simulink model "c00006M_harness"  (R2018a)
settings: Solver=ode3  StartTime=0.0  StopTime=10.0  RelTol=1e-3  EnableMultiTasking=on
undefined symbols (not defined in the file): b, DiscIntNeverNeededParam, J, K, L, PosMinimaW3, R, sigbuilder_block
(part 1 of 42)
settings Model: Creator=aarrieta  LastModifiedBy=umarkiegi
settings DataIOCC: LimitDataPoints=on  SaveFormat=Array
settings OptimizationCC: LifeSpan=inf
settings DebuggingCC: UnderspecifiedInitializationDetection=Classic  MergeDetectMultiDrivingBlocksExec=none  SolverPrmCheckMsg=warning  StateNameClashWarn=warning  SFUnexpectedBacktrackingDiag=warning  SFNoUnconditionalDefaultTransitionDiag=warning  SFExecutionAtInitializationDiag=none
settings HardwareCC: ProdBitPerPointer=32  ProdBitPerSizeT=32  ProdBitPerPtrDiffT=32  ProdLargestAtomicFloat=None  ProdIntDivRoundTo=Undefined  ProdEndianess=Unspecified  ProdWordSize=32  ProdHWDeviceType=32-bit Generic
settings ModelReferenceCC: PropagateSignalLabelsOutOfModel=off
settings CodeAppCC: StateflowObjectComments=on
settings GRTTargetCC: TargetLangStandard=C89/C90 (ANSI)  GeneratePreprocessorConditionals=Disable all
settings ConfigComp: CovMetricSettings=dw  CovHtmlReporting=on  CovSaveCumulativeToWorkspaceVar=on  CovSaveSingleToWorkspaceVar=on  CovExternalEMLEnable=off  DVMaxTestCaseSteps=20  DVTestSuiteOptimization=CombinedObjectives (Nonlinear Extended)  DVDetectFloatOverflow=off

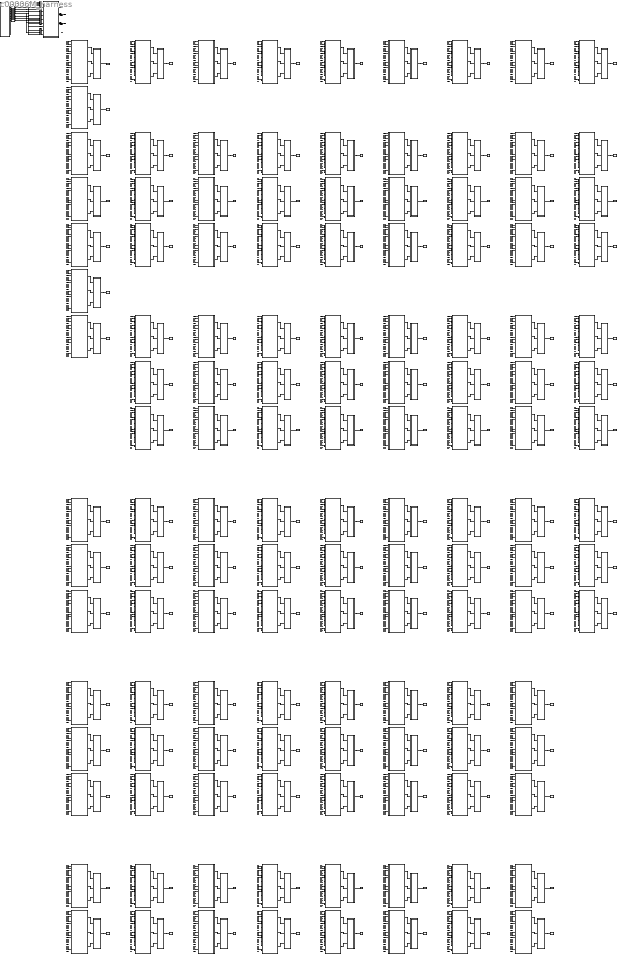
== system c00006M_harness ==
  CPSUT : Subsystem
  Eval : Subsystem
  Eval1 : Subsystem
  Eval10 : Subsystem
  Eval100 : Subsystem
  Eval102 : Subsystem
  Eval103 : Subsystem
  Eval104 : Subsystem
  Eval106 : Subsystem
  Eval107 : Subsystem
  Eval108 : Subsystem
  Eval11 : Subsystem
  Eval110 : Subsystem
  Eval111 : Subsystem
  Eval112 : Subsystem
  Eval114 : Subsystem
  Eval115 : Subsystem
  Eval116 : Subsystem
  Eval118 : Subsystem
  Eval119 : Subsystem
  Eval12 : Subsystem
  Eval120 : Subsystem
  Eval122 : Subsystem
  Eval123 : Subsystem
  Eval124 : Subsystem
  Eval126 : Subsystem
  Eval127 : Subsystem
  Eval128 : Subsystem
  Eval130 : Subsystem
  Eval131 : Subsystem
  Eval132 : Subsystem
  Eval134 : Subsystem
  Eval135 : Subsystem
  Eval136 : Subsystem
  Eval138 : Subsystem
  Eval139 : Subsystem
  Eval14 : Subsystem
  Eval140 : Subsystem
  Eval142 : Subsystem
  Eval143 : Subsystem
  Eval144 : Subsystem
  Eval146 : Subsystem
  Eval147 : Subsystem
  Eval148 : Subsystem
  Eval15 : Subsystem
  Eval150 : Subsystem
  Eval151 : Subsystem
  Eval152 : Subsystem
  Eval154 : Subsystem
  Eval155 : Subsystem
  Eval156 : Subsystem
  Eval158 : Subsystem
  Eval159 : Subsystem
  Eval16 : Subsystem
  Eval160 : Subsystem
  Eval162 : Subsystem
  Eval163 : Subsystem
  Eval164 : Subsystem
  Eval166 : Subsystem
  Eval167 : Subsystem
  Eval168 : Subsystem
  Eval170 : Subsystem
  Eval171 : Subsystem
  Eval172 : Subsystem
  Eval18 : Subsystem
  Eval19 : Subsystem
  Eval2 : Subsystem
  Eval20 : Subsystem
  Eval22 : Subsystem
  Eval23 : Subsystem
  Eval24 : Subsystem
  Eval26 : Subsystem
  Eval27 : Subsystem
  Eval28 : Subsystem
  Eval3 : Subsystem
  Eval30 : Subsystem
  Eval31 : Subsystem
  Eval32 : Subsystem
  Eval34 : Subsystem
  Eval35 : Subsystem
  Eval36 : Subsystem
  Eval38 : Subsystem
  Eval39 : Subsystem
  Eval4 : Subsystem
  Eval40 : Subsystem
  Eval42 : Subsystem
  Eval43 : Subsystem
  Eval44 : Subsystem
  Eval46 : Subsystem
  Eval47 : Subsystem
  Eval48 : Subsystem
  Eval5 : Subsystem
  Eval50 : Subsystem
  Eval51 : Subsystem
  Eval52 : Subsystem
  Eval54 : Subsystem
  Eval55 : Subsystem
  Eval56 : Subsystem
  Eval58 : Subsystem
  Eval59 : Subsystem
  Eval6 : Subsystem
  Eval60 : Subsystem
  Eval62 : Subsystem
  Eval63 : Subsystem
  Eval64 : Subsystem
  Eval66 : Subsystem
  Eval67 : Subsystem
  Eval68 : Subsystem
  Eval70 : Subsystem
  Eval71 : Subsystem
  Eval72 : Subsystem
  Eval74 : Subsystem
  Eval75 : Subsystem
  Eval76 : Subsystem
  Eval78 : Subsystem
  Eval79 : Subsystem
  Eval80 : Subsystem
  Eval82 : Subsystem
  Eval83 : Subsystem
  Eval84 : Subsystem
  Eval86 : Subsystem
  Eval87 : Subsystem
  Eval88 : Subsystem
  Eval90 : Subsystem
  Eval91 : Subsystem
  Eval92 : Subsystem
  Eval94 : Subsystem
  Eval95 : Subsystem
  Eval96 : Subsystem
  Eval98 : Subsystem
  Eval99 : Subsystem
  Inputs : Subsystem  Tag=STV Subsys  LoadFcn=sigbuilder_block('load');  StartFcn=sigbuilder_block('start');  StopFcn=sigbuilder_block('stop');  ClipboardFcn=sigbuilder_block('clipboard');  mask(Sigbuilder block){tuvar=[0:10]}
      mask init:
      | if ~strcmp(get_param(bdroot(gcb),'SimulationStatus'),'stopped'),tuvar = sigbuilder_block('maskInit'); end
      settings: CopyFcn=sigbuilder_block('copy');  DeleteFcn=sigbuilder_block('delete');  ModelCloseFcn=sigbuilder_block('modelClose');  PreSaveFcn=sigbuilder_block('preSave');  PauseFcn=sigbuilder_block('pause');  ContinueFcn=sigbuilder_block('continue');  NameChangeFcn=sigbuilder_block('namechange');  OpenFcn=sigbuilder_block('open');  CloseFcn=sigbuilder_block('close');
      mask Display: plot(0, 0, 100, 100,[2, 2, 32, 32, 2], [68, 8, 8, 68, 68],[32, 2], [38, 38], [32, 19, 2],[53, 60, 44], [32, 17, 17, 2],[16, 16, 31, 31]);txt = getActiveGroup(gcbh);text(2, 100, txt,'verticalAlignment', 'top');
  M001 : Subsystem
  M002 : Subsystem
  M003 : Subsystem
  M004 : Subsystem
  M005 : Subsystem
  M006 : Subsystem
  M007 : Subsystem
  M011 : Subsystem
  M012 : Subsystem
  M013 : Subsystem
  M015 : Subsystem
  M016 : Subsystem
  M017 : Subsystem
  M019 : Subsystem
  M020 : Subsystem
  M021 : Subsystem
  M023 : Subsystem
  M024 : Subsystem
  M025 : Subsystem
  M027 : Subsystem
  M028 : Subsystem
  M029 : Subsystem
  M031 : Subsystem
  M032 : Subsystem
  M033 : Subsystem
  M035 : Subsystem
  M036 : Subsystem
  M037 : Subsystem
  M039 : Subsystem
  M040 : Subsystem
  M041 : Subsystem
  M043 : Subsystem
  M044 : Subsystem
  M045 : Subsystem
  M047 : Subsystem
  M048 : Subsystem
  M049 : Subsystem
  M051 : Subsystem
  M052 : Subsystem
  M053 : Subsystem
  M055 : Subsystem
  M056 : Subsystem
  M057 : Subsystem
  M059 : Subsystem
  M060 : Subsystem
  M061 : Subsystem
  M063 : Subsystem
  M064 : Subsystem
  M065 : Subsystem
  M067 : Subsystem
  M068 : Subsystem
  M069 : Subsystem
  M071 : Subsystem
  M072 : Subsystem
  M073 : Subsystem
  M075 : Subsystem
  M076 : Subsystem
  M077 : Subsystem
  M079 : Subsystem
  M080 : Subsystem
  M081 : Subsystem
  M083 : Subsystem
  M084 : Subsystem
  M085 : Subsystem
  M087 : Subsystem
  M088 : Subsystem
  M089 : Subsystem
  M091 : Subsystem
  M092 : Subsystem
  M093 : Subsystem
  M095 : Subsystem
  M096 : Subsystem
  M097 : Subsystem
  M099 : Subsystem
  M100 : Subsystem
  M101 : Subsystem
  M103 : Subsystem
  M104 : Subsystem
  M105 : Subsystem
  M107 : Subsystem
  M108 : Subsystem
  M109 : Subsystem
  M111 : Subsystem
  M112 : Subsystem
  M113 : Subsystem
  M115 : Subsystem
  M116 : Subsystem
  M117 : Subsystem
  M119 : Subsystem
  M120 : Subsystem
  M121 : Subsystem
  M123 : Subsystem
  M124 : Subsystem
  M125 : Subsystem
  M127 : Subsystem
  M128 : Subsystem
  M129 : Subsystem
  M131 : Subsystem
  M132 : Subsystem
  M133 : Subsystem
  M135 : Subsystem
  M136 : Subsystem
  M137 : Subsystem
  M139 : Subsystem
  M140 : Subsystem
  M141 : Subsystem
  M143 : Subsystem
  M144 : Subsystem
  M145 : Subsystem
  M147 : Subsystem
  M148 : Subsystem
  M149 : Subsystem
  M151 : Subsystem
  M152 : Subsystem
  M153 : Subsystem
  M155 : Subsystem
  M156 : Subsystem
  M157 : Subsystem
  M159 : Subsystem
  M160 : Subsystem
  M161 : Subsystem
  M163 : Subsystem
  M164 : Subsystem
  M165 : Subsystem
  M167 : Subsystem
  M168 : Subsystem
  M169 : Subsystem
  M171 : Subsystem
  M172 : Subsystem
  M173 : Subsystem
  To Workspace : ToWorkspace  VariableName=mutant001  SampleTime=-1
  To Workspace1 : ToWorkspace  VariableName=mutant002  SampleTime=-1
  To Workspace10 : ToWorkspace  VariableName=mutant011  SampleTime=-1
  To Workspace100 : ToWorkspace  VariableName=mutant101  SampleTime=-1
  To Workspace102 : ToWorkspace  VariableName=mutant103  SampleTime=-1
  To Workspace103 : ToWorkspace  VariableName=mutant104  SampleTime=-1
  To Workspace104 : ToWorkspace  VariableName=mutant105  SampleTime=-1
  To Workspace106 : ToWorkspace  VariableName=mutant107  SampleTime=-1
  To Workspace107 : ToWorkspace  VariableName=mutant108  SampleTime=-1
  To Workspace108 : ToWorkspace  VariableName=mutant109  SampleTime=-1
  To Workspace11 : ToWorkspace  VariableName=mutant012  SampleTime=-1
  To Workspace110 : ToWorkspace  VariableName=mutant111  SampleTime=-1
  To Workspace111 : ToWorkspace  VariableName=mutant112  SampleTime=-1
  To Workspace112 : ToWorkspace  VariableName=mutant113  SampleTime=-1
  To Workspace114 : ToWorkspace  VariableName=mutant115  SampleTime=-1
  To Workspace115 : ToWorkspace  VariableName=mutant116  SampleTime=-1
  To Workspace116 : ToWorkspace  VariableName=mutant117  SampleTime=-1
  To Workspace118 : ToWorkspace  VariableName=mutant119  SampleTime=-1
  To Workspace119 : ToWorkspace  VariableName=mutant120  SampleTime=-1
  To Workspace12 : ToWorkspace  VariableName=mutant013  SampleTime=-1
  To Workspace120 : ToWorkspace  VariableName=mutant121  SampleTime=-1
  To Workspace122 : ToWorkspace  VariableName=mutant123  SampleTime=-1
  To Workspace123 : ToWorkspace  VariableName=mutant124  SampleTime=-1
  To Workspace124 : ToWorkspace  VariableName=mutant125  SampleTime=-1
  To Workspace126 : ToWorkspace  VariableName=mutant127  SampleTime=-1
  To Workspace127 : ToWorkspace  VariableName=mutant128  SampleTime=-1
  To Workspace128 : ToWorkspace  VariableName=mutant129  SampleTime=-1
  To Workspace130 : ToWorkspace  VariableName=mutant131  SampleTime=-1
  To Workspace131 : ToWorkspace  VariableName=mutant132  SampleTime=-1
  To Workspace132 : ToWorkspace  VariableName=mutant133  SampleTime=-1
  To Workspace134 : ToWorkspace  VariableName=mutant135  SampleTime=-1
  To Workspace135 : ToWorkspace  VariableName=mutant136  SampleTime=-1
  To Workspace136 : ToWorkspace  VariableName=mutant137  SampleTime=-1
  To Workspace138 : ToWorkspace  VariableName=mutant139  SampleTime=-1
  To Workspace139 : ToWorkspace  VariableName=mutant140  SampleTime=-1
  To Workspace14 : ToWorkspace  VariableName=mutant015  SampleTime=-1
  To Workspace140 : ToWorkspace  VariableName=mutant141  SampleTime=-1
  To Workspace142 : ToWorkspace  VariableName=mutant143  SampleTime=-1
  To Workspace143 : ToWorkspace  VariableName=mutant144  SampleTime=-1
  To Workspace144 : ToWorkspace  VariableName=mutant145  SampleTime=-1
  To Workspace146 : ToWorkspace  VariableName=mutant147  SampleTime=-1
  To Workspace147 : ToWorkspace  VariableName=mutant148  SampleTime=-1
  To Workspace148 : ToWorkspace  VariableName=mutant149  SampleTime=-1
  To Workspace15 : ToWorkspace  VariableName=mutant016  SampleTime=-1
  To Workspace150 : ToWorkspace  VariableName=mutant151  SampleTime=-1
  To Workspace151 : ToWorkspace  VariableName=mutant152  SampleTime=-1
  To Workspace152 : ToWorkspace  VariableName=mutant153  SampleTime=-1
  To Workspace154 : ToWorkspace  VariableName=mutant155  SampleTime=-1
  To Workspace155 : ToWorkspace  VariableName=mutant156  SampleTime=-1
  To Workspace156 : ToWorkspace  VariableName=mutant157  SampleTime=-1
  To Workspace158 : ToWorkspace  VariableName=mutant159  SampleTime=-1
  To Workspace159 : ToWorkspace  VariableName=mutant160  SampleTime=-1
  To Workspace16 : ToWorkspace  VariableName=mutant017  SampleTime=-1
  To Workspace160 : ToWorkspace  VariableName=mutant161  SampleTime=-1
  To Workspace162 : ToWorkspace  VariableName=mutant163  SampleTime=-1
  To Workspace163 : ToWorkspace  VariableName=mutant164  SampleTime=-1
  To Workspace164 : ToWorkspace  VariableName=mutant165  SampleTime=-1
  To Workspace166 : ToWorkspace  VariableName=mutant167  SampleTime=-1
  To Workspace167 : ToWorkspace  VariableName=mutant168  SampleTime=-1
  To Workspace168 : ToWorkspace  VariableName=mutant169  SampleTime=-1
  To Workspace170 : ToWorkspace  VariableName=mutant171  SampleTime=-1
  To Workspace171 : ToWorkspace  VariableName=mutant172  SampleTime=-1
  To Workspace172 : ToWorkspace  VariableName=mutant173  SampleTime=-1
  To Workspace18 : ToWorkspace  VariableName=mutant019  SampleTime=-1
  To Workspace19 : ToWorkspace  VariableName=mutant020  SampleTime=-1
  To Workspace2 : ToWorkspace  VariableName=mutant003  SampleTime=-1
  To Workspace20 : ToWorkspace  VariableName=mutant021  SampleTime=-1
  To Workspace22 : ToWorkspace  VariableName=mutant023  SampleTime=-1
  To Workspace23 : ToWorkspace  VariableName=mutant024  SampleTime=-1
  To Workspace24 : ToWorkspace  VariableName=mutant025  SampleTime=-1
  To Workspace26 : ToWorkspace  VariableName=mutant027  SampleTime=-1
  To Workspace27 : ToWorkspace  VariableName=mutant028  SampleTime=-1
  To Workspace28 : ToWorkspace  VariableName=mutant029  SampleTime=-1
  To Workspace3 : ToWorkspace  VariableName=mutant004  SampleTime=-1
  To Workspace30 : ToWorkspace  VariableName=mutant031  SampleTime=-1
  To Workspace31 : ToWorkspace  VariableName=mutant032  SampleTime=-1
  To Workspace32 : ToWorkspace  VariableName=mutant033  SampleTime=-1
  To Workspace34 : ToWorkspace  VariableName=mutant035  SampleTime=-1
  To Workspace35 : ToWorkspace  VariableName=mutant036  SampleTime=-1
  To Workspace36 : ToWorkspace  VariableName=mutant037  SampleTime=-1
  To Workspace38 : ToWorkspace  VariableName=mutant039  SampleTime=-1
  To Workspace39 : ToWorkspace  VariableName=mutant040  SampleTime=-1
  To Workspace4 : ToWorkspace  VariableName=mutant005  SampleTime=-1
  To Workspace40 : ToWorkspace  VariableName=mutant041  SampleTime=-1
  To Workspace42 : ToWorkspace  VariableName=mutant043  SampleTime=-1
  To Workspace43 : ToWorkspace  VariableName=mutant044  SampleTime=-1
  To Workspace44 : ToWorkspace  VariableName=mutant045  SampleTime=-1
  To Workspace46 : ToWorkspace  VariableName=mutant047  SampleTime=-1
  To Workspace47 : ToWorkspace  VariableName=mutant048  SampleTime=-1
  To Workspace48 : ToWorkspace  VariableName=mutant049  SampleTime=-1
  To Workspace5 : ToWorkspace  VariableName=mutant006  SampleTime=-1
  To Workspace50 : ToWorkspace  VariableName=mutant051  SampleTime=-1
  To Workspace51 : ToWorkspace  VariableName=mutant052  SampleTime=-1
  To Workspace52 : ToWorkspace  VariableName=mutant053  SampleTime=-1
  To Workspace54 : ToWorkspace  VariableName=mutant055  SampleTime=-1
  To Workspace55 : ToWorkspace  VariableName=mutant056  SampleTime=-1
  To Workspace56 : ToWorkspace  VariableName=mutant057  SampleTime=-1
  To Workspace58 : ToWorkspace  VariableName=mutant059  SampleTime=-1
  To Workspace59 : ToWorkspace  VariableName=mutant060  SampleTime=-1
  To Workspace6 : ToWorkspace  VariableName=mutant007  SampleTime=-1
  To Workspace60 : ToWorkspace  VariableName=mutant061  SampleTime=-1
  To Workspace62 : ToWorkspace  VariableName=mutant063  SampleTime=-1
  To Workspace63 : ToWorkspace  VariableName=mutant064  SampleTime=-1
  To Workspace64 : ToWorkspace  VariableName=mutant065  SampleTime=-1
  To Workspace66 : ToWorkspace  VariableName=mutant067  SampleTime=-1
  To Workspace67 : ToWorkspace  VariableName=mutant068  SampleTime=-1
  To Workspace68 : ToWorkspace  VariableName=mutant069  SampleTime=-1
  To Workspace70 : ToWorkspace  VariableName=mutant071  SampleTime=-1
  To Workspace71 : ToWorkspace  VariableName=mutant072  SampleTime=-1
  To Workspace72 : ToWorkspace  VariableName=mutant073  SampleTime=-1
  To Workspace74 : ToWorkspace  VariableName=mutant075  SampleTime=-1
  To Workspace75 : ToWorkspace  VariableName=mutant076  SampleTime=-1
  To Workspace76 : ToWorkspace  VariableName=mutant077  SampleTime=-1
  To Workspace78 : ToWorkspace  VariableName=mutant079  SampleTime=-1
  To Workspace79 : ToWorkspace  VariableName=mutant080  SampleTime=-1
  To Workspace80 : ToWorkspace  VariableName=mutant081  SampleTime=-1
  To Workspace82 : ToWorkspace  VariableName=mutant083  SampleTime=-1
  To Workspace83 : ToWorkspace  VariableName=mutant084  SampleTime=-1
  To Workspace84 : ToWorkspace  VariableName=mutant085  SampleTime=-1
  To Workspace86 : ToWorkspace  VariableName=mutant087  SampleTime=-1
  To Workspace87 : ToWorkspace  VariableName=mutant088  SampleTime=-1
  To Workspace88 : ToWorkspace  VariableName=mutant089  SampleTime=-1
  To Workspace90 : ToWorkspace  VariableName=mutant091  SampleTime=-1
  To Workspace91 : ToWorkspace  VariableName=mutant092  SampleTime=-1
  To Workspace92 : ToWorkspace  VariableName=mutant093  SampleTime=-1
  To Workspace94 : ToWorkspace  VariableName=mutant095  SampleTime=-1
  To Workspace95 : ToWorkspace  VariableName=mutant096  SampleTime=-1
  To Workspace96 : ToWorkspace  VariableName=mutant097  SampleTime=-1
  To Workspace98 : ToWorkspace  VariableName=mutant099  SampleTime=-1
  To Workspace99 : ToWorkspace  VariableName=mutant100  SampleTime=-1
  dtc_CW3C : DataTypeConversion
  dtc_DW1 : DataTypeConversion
  dtc_DW2 : DataTypeConversion
  dtc_DW3 : DataTypeConversion
  dtc_O1 : DataTypeConversion
  dtc_O2 : DataTypeConversion
  dtc_O3 : DataTypeConversion
  dtc_P1W2 : DataTypeConversion
  dtc_P2W3 : DataTypeConversion
  W1Pos : Outport
  W2Pos : Outport  Port=2
  W3Pos : Outport  Port=3
  tag scope: out1=global, out2=global, out3=global, out4=global
  wires:
  CPSUT/2(W2Pos) -> [out2], W2Pos/1
  CPSUT/3(W3Pos) -> W3Pos/1, [out3]
  [in1] -> M001/1(DW1)
  [in2] -> M001/2(DW2)
  [in3] -> M001/3(DW3)
  [in5] -> M001/4(P1W2)
  [in6] -> M001/5(P2W3)
  [in10] -> M001/6(O1)
  [in11] -> M001/7(O2)
  [in12] -> M001/8(O3)
  [in17] -> M001/9(CW3C)
  CPSUT/1(W1Pos) -> [out1], W1Pos/1
  M001/1(W1Pos) -> Eval/1(In1)
  M001/2(W2Pos) -> Eval/2(In2)
  M001/3(W3Pos) -> Eval/3(In3)
  Eval/1(Out1) -> To Workspace/1
  [in1] -> M002/1(DW1)
  [in2] -> M002/2(DW2)
  [in3] -> M002/3(DW3)
  [in5] -> M002/4(P1W2)
  [in6] -> M002/5(P2W3)
  [in10] -> M002/6(O1)
  [in11] -> M002/7(O2)
  [in12] -> M002/8(O3)
  [in17] -> M002/9(CW3C)
  M002/1(W1Pos) -> Eval1/1(In1)
  M002/2(W2Pos) -> Eval1/2(In2)
  M002/3(W3Pos) -> Eval1/3(In3)
  Eval1/1(Out1) -> To Workspace1/1
  [in1] -> M003/1(DW1)
  [in2] -> M003/2(DW2)
  [in3] -> M003/3(DW3)
  [in5] -> M003/4(P1W2)
  [in6] -> M003/5(P2W3)
  [in10] -> M003/6(O1)
  [in11] -> M003/7(O2)
  [in12] -> M003/8(O3)
  [in17] -> M003/9(CW3C)
  M003/1(W1Pos) -> Eval2/1(In1)
  M003/2(W2Pos) -> Eval2/2(In2)
  M003/3(W3Pos) -> Eval2/3(In3)
  Eval2/1(Out1) -> To Workspace2/1
  [in1] -> M004/1(DW1)
  [in2] -> M004/2(DW2)
  [in3] -> M004/3(DW3)
  [in5] -> M004/4(P1W2)
  [in6] -> M004/5(P2W3)
  [in10] -> M004/6(O1)
  [in11] -> M004/7(O2)
  [in12] -> M004/8(O3)
  [in17] -> M004/9(CW3C)
  M004/1(W1Pos) -> Eval3/1(In1)
  M004/2(W2Pos) -> Eval3/2(In2)
  M004/3(W3Pos) -> Eval3/3(In3)
  Eval3/1(Out1) -> To Workspace3/1
  [in1] -> M005/1(DW1)
  [in2] -> M005/2(DW2)
  [in3] -> M005/3(DW3)
  [in5] -> M005/4(P1W2)
  [in6] -> M005/5(P2W3)
  [in10] -> M005/6(O1)
  [in11] -> M005/7(O2)
  [in12] -> M005/8(O3)
  [in17] -> M005/9(CW3C)
  M005/1(W1Pos) -> Eval4/1(In1)
  M005/2(W2Pos) -> Eval4/2(In2)
  M005/3(W3Pos) -> Eval4/3(In3)
  Eval4/1(Out1) -> To Workspace4/1
  [in1] -> M006/1(DW1)
  [in2] -> M006/2(DW2)
  [in3] -> M006/3(DW3)
  [in5] -> M006/4(P1W2)
  [in6] -> M006/5(P2W3)
  [in10] -> M006/6(O1)
  [in11] -> M006/7(O2)
  [in12] -> M006/8(O3)
  [in17] -> M006/9(CW3C)
  M006/1(W1Pos) -> Eval5/1(In1)
  M006/2(W2Pos) -> Eval5/2(In2)
  M006/3(W3Pos) -> Eval5/3(In3)
  Eval5/1(Out1) -> To Workspace5/1
  [in1] -> M007/1(DW1)
  [in2] -> M007/2(DW2)
  [in3] -> M007/3(DW3)
  [in5] -> M007/4(P1W2)
  [in6] -> M007/5(P2W3)
  [in10] -> M007/6(O1)
  [in11] -> M007/7(O2)
  [in12] -> M007/8(O3)
  [in17] -> M007/9(CW3C)
  M007/1(W1Pos) -> Eval6/1(In1)
  M007/2(W2Pos) -> Eval6/2(In2)
  M007/3(W3Pos) -> Eval6/3(In3)
  Eval6/1(Out1) -> To Workspace6/1
  [in1] -> M011/1(DW1)
  [in2] -> M011/2(DW2)
  [in3] -> M011/3(DW3)
  [in5] -> M011/4(P1W2)
  [in6] -> M011/5(P2W3)
  [in10] -> M011/6(O1)
  [in11] -> M011/7(O2)
  [in12] -> M011/8(O3)
  [in17] -> M011/9(CW3C)
  M011/1(W1Pos) -> Eval10/1(In1)
  M011/2(W2Pos) -> Eval10/2(In2)
  M011/3(W3Pos) -> Eval10/3(In3)
  Eval10/1(Out1) -> To Workspace10/1
  [in1] -> M012/1(DW1)
  [in2] -> M012/2(DW2)
  [in3] -> M012/3(DW3)
  [in5] -> M012/4(P1W2)
  [in6] -> M012/5(P2W3)
  [in10] -> M012/6(O1)
  [in11] -> M012/7(O2)
  [in12] -> M012/8(O3)
  [in17] -> M012/9(CW3C)
  M012/1(W1Pos) -> Eval11/1(In1)
  M012/2(W2Pos) -> Eval11/2(In2)
  M012/3(W3Pos) -> Eval11/3(In3)
  Eval11/1(Out1) -> To Workspace11/1
  [in1] -> M013/1(DW1)
  [in2] -> M013/2(DW2)
  [in3] -> M013/3(DW3)
  [in5] -> M013/4(P1W2)
  [in6] -> M013/5(P2W3)
  [in10] -> M013/6(O1)
  [in11] -> M013/7(O2)
  [in12] -> M013/8(O3)
  [in17] -> M013/9(CW3C)
  M013/1(W1Pos) -> Eval12/1(In1)
  M013/2(W2Pos) -> Eval12/2(In2)
  M013/3(W3Pos) -> Eval12/3(In3)
  Eval12/1(Out1) -> To Workspace12/1
  [in1] -> M015/1(DW1)
  [in2] -> M015/2(DW2)
  [in3] -> M015/3(DW3)
  [in5] -> M015/4(P1W2)
  [in6] -> M015/5(P2W3)
  [in10] -> M015/6(O1)
  [in11] -> M015/7(O2)
  [in12] -> M015/8(O3)
  [in17] -> M015/9(CW3C)
  M015/1(W1Pos) -> Eval14/1(In1)
  M015/2(W2Pos) -> Eval14/2(In2)
  M015/3(W3Pos) -> Eval14/3(In3)
  Eval14/1(Out1) -> To Workspace14/1
  [in1] -> M016/1(DW1)
  [in2] -> M016/2(DW2)
  [in3] -> M016/3(DW3)
  [in5] -> M016/4(P1W2)
  [in6] -> M016/5(P2W3)
  [in10] -> M016/6(O1)
  [in11] -> M016/7(O2)
  [in12] -> M016/8(O3)
  [in17] -> M016/9(CW3C)
  M016/1(W1Pos) -> Eval15/1(In1)
  M016/2(W2Pos) -> Eval15/2(In2)
  M016/3(W3Pos) -> Eval15/3(In3)
  Eval15/1(Out1) -> To Workspace15/1
  [in1] -> M017/1(DW1)
  [in2] -> M017/2(DW2)
  [in3] -> M017/3(DW3)
  [in5] -> M017/4(P1W2)
  [in6] -> M017/5(P2W3)
  [in10] -> M017/6(O1)
  [in11] -> M017/7(O2)
  [in12] -> M017/8(O3)
  [in17] -> M017/9(CW3C)
  M017/1(W1Pos) -> Eval16/1(In1)
  M017/2(W2Pos) -> Eval16/2(In2)
  M017/3(W3Pos) -> Eval16/3(In3)
  Eval16/1(Out1) -> To Workspace16/1
  [in1] -> M019/1(DW1)
  [in2] -> M019/2(DW2)
  [in3] -> M019/3(DW3)
  [in5] -> M019/4(P1W2)
  [in6] -> M019/5(P2W3)
  [in10] -> M019/6(O1)
  [in11] -> M019/7(O2)
  [in12] -> M019/8(O3)
  [in17] -> M019/9(CW3C)
  M019/1(W1Pos) -> Eval18/1(In1)
  M019/2(W2Pos) -> Eval18/2(In2)
  M019/3(W3Pos) -> Eval18/3(In3)
  Eval18/1(Out1) -> To Workspace18/1
  [in1] -> M020/1(DW1)
  [in2] -> M020/2(DW2)
  [in3] -> M020/3(DW3)
  [in5] -> M020/4(P1W2)
  [in6] -> M020/5(P2W3)
  [in10] -> M020/6(O1)
  [in11] -> M020/7(O2)
  [in12] -> M020/8(O3)
  [in17] -> M020/9(CW3C)
  M020/1(W1Pos) -> Eval19/1(In1)
  M020/2(W2Pos) -> Eval19/2(In2)
  M020/3(W3Pos) -> Eval19/3(In3)
  Eval19/1(Out1) -> To Workspace19/1
  [in1] -> M021/1(DW1)
  [in2] -> M021/2(DW2)
  [in3] -> M021/3(DW3)
  [in5] -> M021/4(P1W2)
  [in6] -> M021/5(P2W3)
  [in10] -> M021/6(O1)
  [in11] -> M021/7(O2)
  [in12] -> M021/8(O3)
  [in17] -> M021/9(CW3C)
  M021/1(W1Pos) -> Eval20/1(In1)
  M021/2(W2Pos) -> Eval20/2(In2)
  M021/3(W3Pos) -> Eval20/3(In3)
  Eval20/1(Out1) -> To Workspace20/1
  [in1] -> M023/1(DW1)
  [in2] -> M023/2(DW2)
  [in3] -> M023/3(DW3)
  [in5] -> M023/4(P1W2)
  [in6] -> M023/5(P2W3)
  [in10] -> M023/6(O1)
  [in11] -> M023/7(O2)
  [in12] -> M023/8(O3)
  [in17] -> M023/9(CW3C)
  M023/1(W1Pos) -> Eval22/1(In1)
  M023/2(W2Pos) -> Eval22/2(In2)
  M023/3(W3Pos) -> Eval22/3(In3)
  Eval22/1(Out1) -> To Workspace22/1
  [in1] -> M024/1(DW1)
  [in2] -> M024/2(DW2)
  [in3] -> M024/3(DW3)
  [in5] -> M024/4(P1W2)
  [in6] -> M024/5(P2W3)
  [in10] -> M024/6(O1)
  [in11] -> M024/7(O2)
  [in12] -> M024/8(O3)
  [in17] -> M024/9(CW3C)
  M024/1(W1Pos) -> Eval23/1(In1)
  M024/2(W2Pos) -> Eval23/2(In2)
  M024/3(W3Pos) -> Eval23/3(In3)
  Eval23/1(Out1) -> To Workspace23/1
  [in1] -> M025/1(DW1)
  [in2] -> M025/2(DW2)
  [in3] -> M025/3(DW3)
  [in5] -> M025/4(P1W2)
  [in6] -> M025/5(P2W3)
  [in10] -> M025/6(O1)
  [in11] -> M025/7(O2)
  [in12] -> M025/8(O3)
  [in17] -> M025/9(CW3C)
  M025/1(W1Pos) -> Eval24/1(In1)
  M025/2(W2Pos) -> Eval24/2(In2)
  M025/3(W3Pos) -> Eval24/3(In3)
  Eval24/1(Out1) -> To Workspace24/1
  [in1] -> M027/1(DW1)
  [in2] -> M027/2(DW2)
  [in3] -> M027/3(DW3)
  [in5] -> M027/4(P1W2)
  [in6] -> M027/5(P2W3)
  [in10] -> M027/6(O1)
  [in11] -> M027/7(O2)
  [in12] -> M027/8(O3)
  [in17] -> M027/9(CW3C)
  M027/1(W1Pos) -> Eval26/1(In1)
  M027/2(W2Pos) -> Eval26/2(In2)
  M027/3(W3Pos) -> Eval26/3(In3)
  Eval26/1(Out1) -> To Workspace26/1
  [in1] -> M028/1(DW1)
  [in2] -> M028/2(DW2)
  [in3] -> M028/3(DW3)
  [in5] -> M028/4(P1W2)
  [in6] -> M028/5(P2W3)
  [in10] -> M028/6(O1)
  [in11] -> M028/7(O2)
  [in12] -> M028/8(O3)
  [in17] -> M028/9(CW3C)
  M028/1(W1Pos) -> Eval27/1(In1)
  M028/2(W2Pos) -> Eval27/2(In2)
  M028/3(W3Pos) -> Eval27/3(In3)
  Eval27/1(Out1) -> To Workspace27/1
  [in1] -> M029/1(DW1)
  [in2] -> M029/2(DW2)
  [in3] -> M029/3(DW3)
  [in5] -> M029/4(P1W2)
  [in6] -> M029/5(P2W3)
  [in10] -> M029/6(O1)
  [in11] -> M029/7(O2)
  [in12] -> M029/8(O3)
  [in17] -> M029/9(CW3C)
  M029/1(W1Pos) -> Eval28/1(In1)
  M029/2(W2Pos) -> Eval28/2(In2)
  M029/3(W3Pos) -> Eval28/3(In3)
  Eval28/1(Out1) -> To Workspace28/1
  [in1] -> M031/1(DW1)
  [in2] -> M031/2(DW2)
  [in3] -> M031/3(DW3)
  [in5] -> M031/4(P1W2)
  [in6] -> M031/5(P2W3)
  [in10] -> M031/6(O1)
  [in11] -> M031/7(O2)
  [in12] -> M031/8(O3)
  [in17] -> M031/9(CW3C)
  M031/1(W1Pos) -> Eval30/1(In1)
  M031/2(W2Pos) -> Eval30/2(In2)
  M031/3(W3Pos) -> Eval30/3(In3)
  Eval30/1(Out1) -> To Workspace30/1
  [in1] -> M032/1(DW1)
  [in2] -> M032/2(DW2)
  [in3] -> M032/3(DW3)
  [in5] -> M032/4(P1W2)
  [in6] -> M032/5(P2W3)
  [in10] -> M032/6(O1)
  [in11] -> M032/7(O2)
  [in12] -> M032/8(O3)
  [in17] -> M032/9(CW3C)
  M032/1(W1Pos) -> Eval31/1(In1)
  M032/2(W2Pos) -> Eval31/2(In2)
  M032/3(W3Pos) -> Eval31/3(In3)
  Eval31/1(Out1) -> To Workspace31/1
  [in1] -> M033/1(DW1)
  [in2] -> M033/2(DW2)
  [in3] -> M033/3(DW3)
  [in5] -> M033/4(P1W2)
  [in6] -> M033/5(P2W3)
  [in10] -> M033/6(O1)
  [in11] -> M033/7(O2)
  [in12] -> M033/8(O3)
  [in17] -> M033/9(CW3C)
  M033/1(W1Pos) -> Eval32/1(In1)
  M033/2(W2Pos) -> Eval32/2(In2)
  M033/3(W3Pos) -> Eval32/3(In3)
  Eval32/1(Out1) -> To Workspace32/1
  [in1] -> M035/1(DW1)
  [in2] -> M035/2(DW2)
  [in3] -> M035/3(DW3)
  [in5] -> M035/4(P1W2)
  [in6] -> M035/5(P2W3)
  [in10] -> M035/6(O1)
  [in11] -> M035/7(O2)
  [in12] -> M035/8(O3)
  [in17] -> M035/9(CW3C)
  M035/1(W1Pos) -> Eval34/1(In1)
  M035/2(W2Pos) -> Eval34/2(In2)
  M035/3(W3Pos) -> Eval34/3(In3)
  Eval34/1(Out1) -> To Workspace34/1
  [in1] -> M036/1(DW1)
  [in2] -> M036/2(DW2)
  [in3] -> M036/3(DW3)
  [in5] -> M036/4(P1W2)
  [in6] -> M036/5(P2W3)
  [in10] -> M036/6(O1)
  [in11] -> M036/7(O2)
  [in12] -> M036/8(O3)
  [in17] -> M036/9(CW3C)
  M036/1(W1Pos) -> Eval35/1(In1)
  M036/2(W2Pos) -> Eval35/2(In2)
  M036/3(W3Pos) -> Eval35/3(In3)
  Eval35/1(Out1) -> To Workspace35/1
  [in1] -> M037/1(DW1)
  [in2] -> M037/2(DW2)
  [in3] -> M037/3(DW3)
  [in5] -> M037/4(P1W2)
  [in6] -> M037/5(P2W3)
  [in10] -> M037/6(O1)
  [in11] -> M037/7(O2)
  [in12] -> M037/8(O3)
  [in17] -> M037/9(CW3C)
  M037/1(W1Pos) -> Eval36/1(In1)
  M037/2(W2Pos) -> Eval36/2(In2)
  M037/3(W3Pos) -> Eval36/3(In3)
  Eval36/1(Out1) -> To Workspace36/1
  [in1] -> M039/1(DW1)
  [in2] -> M039/2(DW2)
  [in3] -> M039/3(DW3)
  [in5] -> M039/4(P1W2)
  [in6] -> M039/5(P2W3)
  [in10] -> M039/6(O1)
  [in11] -> M039/7(O2)
  [in12] -> M039/8(O3)
  [in17] -> M039/9(CW3C)
  M039/1(W1Pos) -> Eval38/1(In1)
  M039/2(W2Pos) -> Eval38/2(In2)
  M039/3(W3Pos) -> Eval38/3(In3)
  Eval38/1(Out1) -> To Workspace38/1
  [in1] -> M040/1(DW1)
  [in2] -> M040/2(DW2)
  [in3] -> M040/3(DW3)
  [in5] -> M040/4(P1W2)
  [in6] -> M040/5(P2W3)
  [in10] -> M040/6(O1)
  [in11] -> M040/7(O2)
  [in12] -> M040/8(O3)
  [in17] -> M040/9(CW3C)
  M040/1(W1Pos) -> Eval39/1(In1)
  M040/2(W2Pos) -> Eval39/2(In2)
  M040/3(W3Pos) -> Eval39/3(In3)
  Eval39/1(Out1) -> To Workspace39/1
  [in1] -> M041/1(DW1)
  [in2] -> M041/2(DW2)
  [in3] -> M041/3(DW3)
  [in5] -> M041/4(P1W2)
  [in6] -> M041/5(P2W3)
  [in10] -> M041/6(O1)
  [in11] -> M041/7(O2)
  [in12] -> M041/8(O3)
  [in17] -> M041/9(CW3C)
  M041/1(W1Pos) -> Eval40/1(In1)
  M041/2(W2Pos) -> Eval40/2(In2)
  M041/3(W3Pos) -> Eval40/3(In3)
  Eval40/1(Out1) -> To Workspace40/1
  [in1] -> M043/1(DW1)
  [in2] -> M043/2(DW2)
  [in3] -> M043/3(DW3)
  [in5] -> M043/4(P1W2)
  [in6] -> M043/5(P2W3)
  [in10] -> M043/6(O1)
  [in11] -> M043/7(O2)
  [in12] -> M043/8(O3)
  [in17] -> M043/9(CW3C)
  M043/1(W1Pos) -> Eval42/1(In1)
  M043/2(W2Pos) -> Eval42/2(In2)
  M043/3(W3Pos) -> Eval42/3(In3)
  Eval42/1(Out1) -> To Workspace42/1
  [in1] -> M044/1(DW1)
  [in2] -> M044/2(DW2)
  [in3] -> M044/3(DW3)
  [in5] -> M044/4(P1W2)
  [in6] -> M044/5(P2W3)
  [in10] -> M044/6(O1)
  [in11] -> M044/7(O2)
  [in12] -> M044/8(O3)
  [in17] -> M044/9(CW3C)
  M044/1(W1Pos) -> Eval43/1(In1)
  M044/2(W2Pos) -> Eval43/2(In2)
  M044/3(W3Pos) -> Eval43/3(In3)
  Eval43/1(Out1) -> To Workspace43/1
  [in1] -> M045/1(DW1)
  [in2] -> M045/2(DW2)
  [in3] -> M045/3(DW3)
  [in5] -> M045/4(P1W2)
  [in6] -> M045/5(P2W3)
  [in10] -> M045/6(O1)
  [in11] -> M045/7(O2)
  [in12] -> M045/8(O3)
  [in17] -> M045/9(CW3C)
  M045/1(W1Pos) -> Eval44/1(In1)
  M045/2(W2Pos) -> Eval44/2(In2)
  M045/3(W3Pos) -> Eval44/3(In3)
  Eval44/1(Out1) -> To Workspace44/1
  [in1] -> M047/1(DW1)
  [in2] -> M047/2(DW2)
  [in3] -> M047/3(DW3)
  [in5] -> M047/4(P1W2)
  [in6] -> M047/5(P2W3)
  [in10] -> M047/6(O1)
  [in11] -> M047/7(O2)
  [in12] -> M047/8(O3)
  [in17] -> M047/9(CW3C)
  M047/1(W1Pos) -> Eval46/1(In1)
  M047/2(W2Pos) -> Eval46/2(In2)
  M047/3(W3Pos) -> Eval46/3(In3)
  Eval46/1(Out1) -> To Workspace46/1
  [in1] -> M048/1(DW1)
  [in2] -> M048/2(DW2)
  [in3] -> M048/3(DW3)
  [in5] -> M048/4(P1W2)
  [in6] -> M048/5(P2W3)
  [in10] -> M048/6(O1)
  [in11] -> M048/7(O2)
  [in12] -> M048/8(O3)
  [in17] -> M048/9(CW3C)
  M048/1(W1Pos) -> Eval47/1(In1)
  M048/2(W2Pos) -> Eval47/2(In2)
  M048/3(W3Pos) -> Eval47/3(In3)
  Eval47/1(Out1) -> To Workspace47/1
  [in1] -> M049/1(DW1)
  [in2] -> M049/2(DW2)
  [in3] -> M049/3(DW3)
  [in5] -> M049/4(P1W2)
  [in6] -> M049/5(P2W3)
  [in10] -> M049/6(O1)
  [in11] -> M049/7(O2)
  [in12] -> M049/8(O3)
  [in17] -> M049/9(CW3C)
  M049/1(W1Pos) -> Eval48/1(In1)
  M049/2(W2Pos) -> Eval48/2(In2)
  M049/3(W3Pos) -> Eval48/3(In3)
  Eval48/1(Out1) -> To Workspace48/1
  [in1] -> M051/1(DW1)
  [in2] -> M051/2(DW2)
  [in3] -> M051/3(DW3)
  [in5] -> M051/4(P1W2)
  [in6] -> M051/5(P2W3)
  [in10] -> M051/6(O1)
  [in11] -> M051/7(O2)
  [in12] -> M051/8(O3)
  [in17] -> M051/9(CW3C)
  M051/1(W1Pos) -> Eval50/1(In1)
  M051/2(W2Pos) -> Eval50/2(In2)
  M051/3(W3Pos) -> Eval50/3(In3)
  Eval50/1(Out1) -> To Workspace50/1
  [in1] -> M052/1(DW1)
  [in2] -> M052/2(DW2)
  [in3] -> M052/3(DW3)
  [in5] -> M052/4(P1W2)
  [in6] -> M052/5(P2W3)
  [in10] -> M052/6(O1)
  [in11] -> M052/7(O2)
  [in12] -> M052/8(O3)
  [in17] -> M052/9(CW3C)
  M052/1(W1Pos) -> Eval51/1(In1)
  M052/2(W2Pos) -> Eval51/2(In2)
  M052/3(W3Pos) -> Eval51/3(In3)
  Eval51/1(Out1) -> To Workspace51/1
  [in1] -> M053/1(DW1)
  [in2] -> M053/2(DW2)
  [in3] -> M053/3(DW3)
  [in5] -> M053/4(P1W2)
  [in6] -> M053/5(P2W3)
  [in10] -> M053/6(O1)
  [in11] -> M053/7(O2)
  [in12] -> M053/8(O3)
  [in17] -> M053/9(CW3C)
  M053/1(W1Pos) -> Eval52/1(In1)
  M053/2(W2Pos) -> Eval52/2(In2)
  M053/3(W3Pos) -> Eval52/3(In3)
  Eval52/1(Out1) -> To Workspace52/1
  [in1] -> M055/1(DW1)
  [in2] -> M055/2(DW2)
  [in3] -> M055/3(DW3)
  [in5] -> M055/4(P1W2)
  [in6] -> M055/5(P2W3)
  [in10] -> M055/6(O1)
  [in11] -> M055/7(O2)
  [in12] -> M055/8(O3)
  [in17] -> M055/9(CW3C)
  M055/1(W1Pos) -> Eval54/1(In1)
  M055/2(W2Pos) -> Eval54/2(In2)
  M055/3(W3Pos) -> Eval54/3(In3)
  Eval54/1(Out1) -> To Workspace54/1
  [in1] -> M056/1(DW1)
  [in2] -> M056/2(DW2)
  [in3] -> M056/3(DW3)
  [in5] -> M056/4(P1W2)
  [in6] -> M056/5(P2W3)
  [in10] -> M056/6(O1)
  [in11] -> M056/7(O2)
  [in12] -> M056/8(O3)
  [in17] -> M056/9(CW3C)
  M056/1(W1Pos) -> Eval55/1(In1)
  M056/2(W2Pos) -> Eval55/2(In2)
  M056/3(W3Pos) -> Eval55/3(In3)
  Eval55/1(Out1) -> To Workspace55/1
  [in1] -> M057/1(DW1)
  [in2] -> M057/2(DW2)
  [in3] -> M057/3(DW3)
  [in5] -> M057/4(P1W2)
  [in6] -> M057/5(P2W3)
  [in10] -> M057/6(O1)
  [in11] -> M057/7(O2)
  [in12] -> M057/8(O3)
  [in17] -> M057/9(CW3C)
  M057/1(W1Pos) -> Eval56/1(In1)
  M057/2(W2Pos) -> Eval56/2(In2)
  M057/3(W3Pos) -> Eval56/3(In3)
  Eval56/1(Out1) -> To Workspace56/1
  [in1] -> M059/1(DW1)
  [in2] -> M059/2(DW2)
  [in3] -> M059/3(DW3)
  [in5] -> M059/4(P1W2)
  [in6] -> M059/5(P2W3)
  [in10] -> M059/6(O1)
  [in11] -> M059/7(O2)
  [in12] -> M059/8(O3)
  [in17] -> M059/9(CW3C)
  M059/1(W1Pos) -> Eval58/1(In1)
  M059/2(W2Pos) -> Eval58/2(In2)
  M059/3(W3Pos) -> Eval58/3(In3)
  Eval58/1(Out1) -> To Workspace58/1
  [in1] -> M060/1(DW1)
  [in2] -> M060/2(DW2)
  [in3] -> M060/3(DW3)
  [in5] -> M060/4(P1W2)
  [in6] -> M060/5(P2W3)
  [in10] -> M060/6(O1)
  [in11] -> M060/7(O2)
  [in12] -> M060/8(O3)
  [in17] -> M060/9(CW3C)
  M060/1(W1Pos) -> Eval59/1(In1)
  M060/2(W2Pos) -> Eval59/2(In2)
  M060/3(W3Pos) -> Eval59/3(In3)
  Eval59/1(Out1) -> To Workspace59/1
  [in1] -> M061/1(DW1)
  [in2] -> M061/2(DW2)
  [in3] -> M061/3(DW3)
  [in5] -> M061/4(P1W2)
  [in6] -> M061/5(P2W3)
  [in10] -> M061/6(O1)
  [in11] -> M061/7(O2)
  [in12] -> M061/8(O3)
  [in17] -> M061/9(CW3C)
  M061/1(W1Pos) -> Eval60/1(In1)
  M061/2(W2Pos) -> Eval60/2(In2)
  M061/3(W3Pos) -> Eval60/3(In3)
  Eval60/1(Out1) -> To Workspace60/1
  [in1] -> M063/1(DW1)
  [in2] -> M063/2(DW2)
  [in3] -> M063/3(DW3)
  [in5] -> M063/4(P1W2)
  [in6] -> M063/5(P2W3)
  [in10] -> M063/6(O1)
  [in11] -> M063/7(O2)
  [in12] -> M063/8(O3)
  [in17] -> M063/9(CW3C)
  M063/1(W1Pos) -> Eval62/1(In1)
  M063/2(W2Pos) -> Eval62/2(In2)
  M063/3(W3Pos) -> Eval62/3(In3)
  Eval62/1(Out1) -> To Workspace62/1
  [in1] -> M064/1(DW1)
  [in2] -> M064/2(DW2)
  [in3] -> M064/3(DW3)
  [in5] -> M064/4(P1W2)
  [in6] -> M064/5(P2W3)
  [in10] -> M064/6(O1)
  [in11] -> M064/7(O2)
  [in12] -> M064/8(O3)
  [in17] -> M064/9(CW3C)
  M064/1(W1Pos) -> Eval63/1(In1)
  M064/2(W2Pos) -> Eval63/2(In2)
  M064/3(W3Pos) -> Eval63/3(In3)
  Eval63/1(Out1) -> To Workspace63/1
  [in1] -> M065/1(DW1)
  [in2] -> M065/2(DW2)
  [in3] -> M065/3(DW3)
  [in5] -> M065/4(P1W2)
  [in6] -> M065/5(P2W3)
  [in10] -> M065/6(O1)
  [in11] -> M065/7(O2)
  [in12] -> M065/8(O3)
  [in17] -> M065/9(CW3C)
  M065/1(W1Pos) -> Eval64/1(In1)
  M065/2(W2Pos) -> Eval64/2(In2)
  M065/3(W3Pos) -> Eval64/3(In3)
  Eval64/1(Out1) -> To Workspace64/1
  [in1] -> M067/1(DW1)
  [in2] -> M067/2(DW2)
  [in3] -> M067/3(DW3)
  [in5] -> M067/4(P1W2)
  [in6] -> M067/5(P2W3)
  [in10] -> M067/6(O1)
  [in11] -> M067/7(O2)
  [in12] -> M067/8(O3)
  [in17] -> M067/9(CW3C)
  M067/1(W1Pos) -> Eval66/1(In1)
  M067/2(W2Pos) -> Eval66/2(In2)
  M067/3(W3Pos) -> Eval66/3(In3)
  Eval66/1(Out1) -> To Workspace66/1
  [in1] -> M068/1(DW1)
  [in2] -> M068/2(DW2)
  [in3] -> M068/3(DW3)
  [in5] -> M068/4(P1W2)
  [in6] -> M068/5(P2W3)
  [in10] -> M068/6(O1)
  [in11] -> M068/7(O2)
  [in12] -> M068/8(O3)
  [in17] -> M068/9(CW3C)
  M068/1(W1Pos) -> Eval67/1(In1)
  M068/2(W2Pos) -> Eval67/2(In2)
  M068/3(W3Pos) -> Eval67/3(In3)
  Eval67/1(Out1) -> To Workspace67/1
  [in1] -> M069/1(DW1)
  [in2] -> M069/2(DW2)
  [in3] -> M069/3(DW3)
  [in5] -> M069/4(P1W2)
  [in6] -> M069/5(P2W3)
  [in10] -> M069/6(O1)
  [in11] -> M069/7(O2)
  [in12] -> M069/8(O3)
  [in17] -> M069/9(CW3C)
  M069/1(W1Pos) -> Eval68/1(In1)
  M069/2(W2Pos) -> Eval68/2(In2)
  M069/3(W3Pos) -> Eval68/3(In3)
  Eval68/1(Out1) -> To Workspace68/1
  [in1] -> M071/1(DW1)
  [in2] -> M071/2(DW2)
  [in3] -> M071/3(DW3)
  [in5] -> M071/4(P1W2)
  [in6] -> M071/5(P2W3)
  [in10] -> M071/6(O1)
  [in11] -> M071/7(O2)
  [in12] -> M071/8(O3)
  [in17] -> M071/9(CW3C)
  M071/1(W1Pos) -> Eval70/1(In1)
  M071/2(W2Pos) -> Eval70/2(In2)
  M071/3(W3Pos) -> Eval70/3(In3)
  Eval70/1(Out1) -> To Workspace70/1
  [in1] -> M072/1(DW1)
  [in2] -> M072/2(DW2)
  [in3] -> M072/3(DW3)
  [in5] -> M072/4(P1W2)
  [in6] -> M072/5(P2W3)
  [in10] -> M072/6(O1)
  [in11] -> M072/7(O2)
  [in12] -> M072/8(O3)
  [in17] -> M072/9(CW3C)
  M072/1(W1Pos) -> Eval71/1(In1)
  M072/2(W2Pos) -> Eval71/2(In2)
  M072/3(W3Pos) -> Eval71/3(In3)
  Eval71/1(Out1) -> To Workspace71/1
  [in1] -> M073/1(DW1)
  [in2] -> M073/2(DW2)
  [in3] -> M073/3(DW3)
  [in5] -> M073/4(P1W2)
  [in6] -> M073/5(P2W3)
  [in10] -> M073/6(O1)
  [in11] -> M073/7(O2)
  [in12] -> M073/8(O3)
  [in17] -> M073/9(CW3C)
  M073/1(W1Pos) -> Eval72/1(In1)
  M073/2(W2Pos) -> Eval72/2(In2)
  M073/3(W3Pos) -> Eval72/3(In3)
  Eval72/1(Out1) -> To Workspace72/1
  [in1] -> M075/1(DW1)
  [in2] -> M075/2(DW2)
  [in3] -> M075/3(DW3)
  [in5] -> M075/4(P1W2)
  [in6] -> M075/5(P2W3)
  [in10] -> M075/6(O1)
  [in11] -> M075/7(O2)
  [in12] -> M075/8(O3)
  [in17] -> M075/9(CW3C)
  M075/1(W1Pos) -> Eval74/1(In1)
  M075/2(W2Pos) -> Eval74/2(In2)
  M075/3(W3Pos) -> Eval74/3(In3)
  Eval74/1(Out1) -> To Workspace74/1
  [in1] -> M076/1(DW1)
  [in2] -> M076/2(DW2)
  [in3] -> M076/3(DW3)
  [in5] -> M076/4(P1W2)
  [in6] -> M076/5(P2W3)
  [in10] -> M076/6(O1)
  [in11] -> M076/7(O2)
  [in12] -> M076/8(O3)
  [in17] -> M076/9(CW3C)
  M076/1(W1Pos) -> Eval75/1(In1)
  M076/2(W2Pos) -> Eval75/2(In2)
  M076/3(W3Pos) -> Eval75/3(In3)
  Eval75/1(Out1) -> To Workspace75/1
  [in1] -> M077/1(DW1)
  [in2] -> M077/2(DW2)
  [in3] -> M077/3(DW3)
  [in5] -> M077/4(P1W2)
  [in6] -> M077/5(P2W3)
  [in10] -> M077/6(O1)
  [in11] -> M077/7(O2)
  [in12] -> M077/8(O3)
  [in17] -> M077/9(CW3C)
  M077/1(W1Pos) -> Eval76/1(In1)
  M077/2(W2Pos) -> Eval76/2(In2)
  M077/3(W3Pos) -> Eval76/3(In3)
  Eval76/1(Out1) -> To Workspace76/1
  [in1] -> M079/1(DW1)
  [in2] -> M079/2(DW2)
  [in3] -> M079/3(DW3)
  [in5] -> M079/4(P1W2)
  [in6] -> M079/5(P2W3)
  [in10] -> M079/6(O1)
  [in11] -> M079/7(O2)
  [in12] -> M079/8(O3)
  [in17] -> M079/9(CW3C)
  M079/1(W1Pos) -> Eval78/1(In1)
  M079/2(W2Pos) -> Eval78/2(In2)
  M079/3(W3Pos) -> Eval78/3(In3)
  Eval78/1(Out1) -> To Workspace78/1
  [in1] -> M080/1(DW1)
  [in2] -> M080/2(DW2)
  [in3] -> M080/3(DW3)
  [in5] -> M080/4(P1W2)
  [in6] -> M080/5(P2W3)
  [in10] -> M080/6(O1)
  [in11] -> M080/7(O2)
  [in12] -> M080/8(O3)
  [in17] -> M080/9(CW3C)
  M080/1(W1Pos) -> Eval79/1(In1)
  M080/2(W2Pos) -> Eval79/2(In2)
  M080/3(W3Pos) -> Eval79/3(In3)
  Eval79/1(Out1) -> To Workspace79/1
  [in1] -> M081/1(DW1)
  [in2] -> M081/2(DW2)
  [in3] -> M081/3(DW3)
  [in5] -> M081/4(P1W2)
  [in6] -> M081/5(P2W3)
  [in10] -> M081/6(O1)
  [in11] -> M081/7(O2)
  [in12] -> M081/8(O3)
  [in17] -> M081/9(CW3C)
  M081/1(W1Pos) -> Eval80/1(In1)
  M081/2(W2Pos) -> Eval80/2(In2)
  M081/3(W3Pos) -> Eval80/3(In3)
  Eval80/1(Out1) -> To Workspace80/1
  [in1] -> M083/1(DW1)
  [in2] -> M083/2(DW2)
  [in3] -> M083/3(DW3)
  [in5] -> M083/4(P1W2)
  [in6] -> M083/5(P2W3)
  [in10] -> M083/6(O1)
  [in11] -> M083/7(O2)
  [in12] -> M083/8(O3)
  [in17] -> M083/9(CW3C)
  M083/1(W1Pos) -> Eval82/1(In1)
  M083/2(W2Pos) -> Eval82/2(In2)
  M083/3(W3Pos) -> Eval82/3(In3)
  Eval82/1(Out1) -> To Workspace82/1
  [in1] -> M084/1(DW1)
  [in2] -> M084/2(DW2)
  [in3] -> M084/3(DW3)
  [in5] -> M084/4(P1W2)
  [in6] -> M084/5(P2W3)
  [in10] -> M084/6(O1)
  [in11] -> M084/7(O2)
  [in12] -> M084/8(O3)
  [in17] -> M084/9(CW3C)
  M084/1(W1Pos) -> Eval83/1(In1)
  M084/2(W2Pos) -> Eval83/2(In2)
  M084/3(W3Pos) -> Eval83/3(In3)
  Eval83/1(Out1) -> To Workspace83/1
  [in1] -> M085/1(DW1)
  [in2] -> M085/2(DW2)
  [in3] -> M085/3(DW3)
  [in5] -> M085/4(P1W2)
  [in6] -> M085/5(P2W3)
  [in10] -> M085/6(O1)
  [in11] -> M085/7(O2)
  [in12] -> M085/8(O3)
  [in17] -> M085/9(CW3C)
  M085/1(W1Pos) -> Eval84/1(In1)
  M085/2(W2Pos) -> Eval84/2(In2)
  M085/3(W3Pos) -> Eval84/3(In3)
  Eval84/1(Out1) -> To Workspace84/1
  [in1] -> M087/1(DW1)
  [in2] -> M087/2(DW2)
  [in3] -> M087/3(DW3)
  [in5] -> M087/4(P1W2)
  [in6] -> M087/5(P2W3)
  [in10] -> M087/6(O1)
  [in11] -> M087/7(O2)
  [in12] -> M087/8(O3)
  [in17] -> M087/9(CW3C)
  M087/1(W1Pos) -> Eval86/1(In1)
  M087/2(W2Pos) -> Eval86/2(In2)
  M087/3(W3Pos) -> Eval86/3(In3)
  Eval86/1(Out1) -> To Workspace86/1
  [in1] -> M088/1(DW1)
  [in2] -> M088/2(DW2)
  [in3] -> M088/3(DW3)
  [in5] -> M088/4(P1W2)
  [in6] -> M088/5(P2W3)
  [in10] -> M088/6(O1)
  [in11] -> M088/7(O2)
  [in12] -> M088/8(O3)
  [in17] -> M088/9(CW3C)
  M088/1(W1Pos) -> Eval87/1(In1)
  M088/2(W2Pos) -> Eval87/2(In2)
  M088/3(W3Pos) -> Eval87/3(In3)
  Eval87/1(Out1) -> To Workspace87/1
  [in1] -> M089/1(DW1)
  [in2] -> M089/2(DW2)
  [in3] -> M089/3(DW3)
  [in5] -> M089/4(P1W2)
  [in6] -> M089/5(P2W3)
  [in10] -> M089/6(O1)
  [in11] -> M089/7(O2)
  [in12] -> M089/8(O3)
  [in17] -> M089/9(CW3C)
  M089/1(W1Pos) -> Eval88/1(In1)
  M089/2(W2Pos) -> Eval88/2(In2)
  M089/3(W3Pos) -> Eval88/3(In3)
  Eval88/1(Out1) -> To Workspace88/1
  [in1] -> M091/1(DW1)
  [in2] -> M091/2(DW2)
  [in3] -> M091/3(DW3)
  [in5] -> M091/4(P1W2)
  [in6] -> M091/5(P2W3)
  [in10] -> M091/6(O1)
  [in11] -> M091/7(O2)
  [in12] -> M091/8(O3)
  [in17] -> M091/9(CW3C)
  M091/1(W1Pos) -> Eval90/1(In1)
  M091/2(W2Pos) -> Eval90/2(In2)
  M091/3(W3Pos) -> Eval90/3(In3)
  Eval90/1(Out1) -> To Workspace90/1
  [in1] -> M092/1(DW1)
  [in2] -> M092/2(DW2)
  [in3] -> M092/3(DW3)
  [in5] -> M092/4(P1W2)
  [in6] -> M092/5(P2W3)
  [in10] -> M092/6(O1)
  [in11] -> M092/7(O2)
  [in12] -> M092/8(O3)
  [in17] -> M092/9(CW3C)
  M092/1(W1Pos) -> Eval91/1(In1)
  M092/2(W2Pos) -> Eval91/2(In2)
  M092/3(W3Pos) -> Eval91/3(In3)
  Eval91/1(Out1) -> To Workspace91/1
  [in1] -> M093/1(DW1)
  [in2] -> M093/2(DW2)
  [in3] -> M093/3(DW3)
  [in5] -> M093/4(P1W2)
  [in6] -> M093/5(P2W3)
  [in10] -> M093/6(O1)
  [in11] -> M093/7(O2)
  [in12] -> M093/8(O3)
  [in17] -> M093/9(CW3C)
  M093/1(W1Pos) -> Eval92/1(In1)
  M093/2(W2Pos) -> Eval92/2(In2)
  M093/3(W3Pos) -> Eval92/3(In3)
  Eval92/1(Out1) -> To Workspace92/1
  [in1] -> M095/1(DW1)
  [in2] -> M095/2(DW2)
  [in3] -> M095/3(DW3)
  [in5] -> M095/4(P1W2)
  [in6] -> M095/5(P2W3)
  [in10] -> M095/6(O1)
  [in11] -> M095/7(O2)
  [in12] -> M095/8(O3)
  [in17] -> M095/9(CW3C)
  M095/1(W1Pos) -> Eval94/1(In1)
  M095/2(W2Pos) -> Eval94/2(In2)
  M095/3(W3Pos) -> Eval94/3(In3)
  Eval94/1(Out1) -> To Workspace94/1
  [in1] -> M096/1(DW1)
  [in2] -> M096/2(DW2)
  [in3] -> M096/3(DW3)
  [in5] -> M096/4(P1W2)
  [in6] -> M096/5(P2W3)
  [in10] -> M096/6(O1)
  [in11] -> M096/7(O2)
  [in12] -> M096/8(O3)
  [in17] -> M096/9(CW3C)
  M096/1(W1Pos) -> Eval95/1(In1)
  M096/2(W2Pos) -> Eval95/2(In2)
  M096/3(W3Pos) -> Eval95/3(In3)
  Eval95/1(Out1) -> To Workspace95/1
  [in1] -> M097/1(DW1)
  [in2] -> M097/2(DW2)
  [in3] -> M097/3(DW3)
  [in5] -> M097/4(P1W2)
  [in6] -> M097/5(P2W3)
  [in10] -> M097/6(O1)
  [in11] -> M097/7(O2)
  [in12] -> M097/8(O3)
  [in17] -> M097/9(CW3C)
  M097/1(W1Pos) -> Eval96/1(In1)
  M097/2(W2Pos) -> Eval96/2(In2)
  M097/3(W3Pos) -> Eval96/3(In3)
  Eval96/1(Out1) -> To Workspace96/1
  [in1] -> M099/1(DW1)
  [in2] -> M099/2(DW2)
  [in3] -> M099/3(DW3)
  [in5] -> M099/4(P1W2)
  [in6] -> M099/5(P2W3)
  [in10] -> M099/6(O1)
  [in11] -> M099/7(O2)
  [in12] -> M099/8(O3)
  [in17] -> M099/9(CW3C)
  M099/1(W1Pos) -> Eval98/1(In1)
  M099/2(W2Pos) -> Eval98/2(In2)
  M099/3(W3Pos) -> Eval98/3(In3)
  Eval98/1(Out1) -> To Workspace98/1
  [in1] -> M100/1(DW1)
  [in2] -> M100/2(DW2)
  [in3] -> M100/3(DW3)
  [in5] -> M100/4(P1W2)
  [in6] -> M100/5(P2W3)
  [in10] -> M100/6(O1)
  [in11] -> M100/7(O2)
  [in12] -> M100/8(O3)
  [in17] -> M100/9(CW3C)
  M100/1(W1Pos) -> Eval99/1(In1)
  M100/2(W2Pos) -> Eval99/2(In2)
  M100/3(W3Pos) -> Eval99/3(In3)
  Eval99/1(Out1) -> To Workspace99/1
  [in1] -> M101/1(DW1)
  [in2] -> M101/2(DW2)
  [in3] -> M101/3(DW3)
  [in5] -> M101/4(P1W2)
  [in6] -> M101/5(P2W3)
  [in10] -> M101/6(O1)
  [in11] -> M101/7(O2)
  [in12] -> M101/8(O3)
  [in17] -> M101/9(CW3C)
  M101/1(W1Pos) -> Eval100/1(In1)
  M101/2(W2Pos) -> Eval100/2(In2)
  M101/3(W3Pos) -> Eval100/3(In3)
  Eval100/1(Out1) -> To Workspace100/1
  [in1] -> M103/1(DW1)
  [in2] -> M103/2(DW2)
  [in3] -> M103/3(DW3)
  [in5] -> M103/4(P1W2)
  [in6] -> M103/5(P2W3)
  [in10] -> M103/6(O1)
  [in11] -> M103/7(O2)
  [in12] -> M103/8(O3)
  [in17] -> M103/9(CW3C)
  M103/1(W1Pos) -> Eval102/1(In1)
  M103/2(W2Pos) -> Eval102/2(In2)
  M103/3(W3Pos) -> Eval102/3(In3)
  Eval102/1(Out1) -> To Workspace102/1
  [in1] -> M104/1(DW1)
  [in2] -> M104/2(DW2)
  [in3] -> M104/3(DW3)
  [in5] -> M104/4(P1W2)
  [in6] -> M104/5(P2W3)
  [in10] -> M104/6(O1)
  [in11] -> M104/7(O2)
  [in12] -> M104/8(O3)
  [in17] -> M104/9(CW3C)
  M104/1(W1Pos) -> Eval103/1(In1)
  M104/2(W2Pos) -> Eval103/2(In2)
  M104/3(W3Pos) -> Eval103/3(In3)
  Eval103/1(Out1) -> To Workspace103/1
  [in1] -> M105/1(DW1)
  [in2] -> M105/2(DW2)
  [in3] -> M105/3(DW3)
  [in5] -> M105/4(P1W2)
  [in6] -> M105/5(P2W3)
  [in10] -> M105/6(O1)
  [in11] -> M105/7(O2)
  [in12] -> M105/8(O3)
  [in17] -> M105/9(CW3C)
  M105/1(W1Pos) -> Eval104/1(In1)
  M105/2(W2Pos) -> Eval104/2(In2)
  M105/3(W3Pos) -> Eval104/3(In3)
  Eval104/1(Out1) -> To Workspace104/1
  [in1] -> M107/1(DW1)
  [in2] -> M107/2(DW2)
  [in3] -> M107/3(DW3)
  [in5] -> M107/4(P1W2)
  [in6] -> M107/5(P2W3)
  [in10] -> M107/6(O1)
  [in11] -> M107/7(O2)
  [in12] -> M107/8(O3)
  [in17] -> M107/9(CW3C)
  M107/1(W1Pos) -> Eval106/1(In1)
  M107/2(W2Pos) -> Eval106/2(In2)
  M107/3(W3Pos) -> Eval106/3(In3)
  Eval106/1(Out1) -> To Workspace106/1
  [in1] -> M108/1(DW1)
  [in2] -> M108/2(DW2)
  [in3] -> M108/3(DW3)
  [in5] -> M108/4(P1W2)
  [in6] -> M108/5(P2W3)
  [in10] -> M108/6(O1)
  [in11] -> M108/7(O2)
  [in12] -> M108/8(O3)
  [in17] -> M108/9(CW3C)
  M108/1(W1Pos) -> Eval107/1(In1)
  M108/2(W2Pos) -> Eval107/2(In2)
  M108/3(W3Pos) -> Eval107/3(In3)
  Eval107/1(Out1) -> To Workspace107/1
  [in1] -> M109/1(DW1)
  [in2] -> M109/2(DW2)
  [in3] -> M109/3(DW3)
  [in5] -> M109/4(P1W2)
  [in6] -> M109/5(P2W3)
  [in10] -> M109/6(O1)
  [in11] -> M109/7(O2)
  [in12] -> M109/8(O3)
  [in17] -> M109/9(CW3C)
  M109/1(W1Pos) -> Eval108/1(In1)
  M109/2(W2Pos) -> Eval108/2(In2)
  M109/3(W3Pos) -> Eval108/3(In3)
  Eval108/1(Out1) -> To Workspace108/1
  [in1] -> M111/1(DW1)
  [in2] -> M111/2(DW2)
  [in3] -> M111/3(DW3)
  [in5] -> M111/4(P1W2)
  [in6] -> M111/5(P2W3)
  [in10] -> M111/6(O1)
  [in11] -> M111/7(O2)
  [in12] -> M111/8(O3)
  [in17] -> M111/9(CW3C)
  M111/1(W1Pos) -> Eval110/1(In1)
  M111/2(W2Pos) -> Eval110/2(In2)
  M111/3(W3Pos) -> Eval110/3(In3)
  Eval110/1(Out1) -> To Workspace110/1
  [in1] -> M112/1(DW1)
  [in2] -> M112/2(DW2)
  [in3] -> M112/3(DW3)
  [in5] -> M112/4(P1W2)
  [in6] -> M112/5(P2W3)
  [in10] -> M112/6(O1)
  [in11] -> M112/7(O2)
  [in12] -> M112/8(O3)
  [in17] -> M112/9(CW3C)
  M112/1(W1Pos) -> Eval111/1(In1)
  M112/2(W2Pos) -> Eval111/2(In2)
  M112/3(W3Pos) -> Eval111/3(In3)
  Eval111/1(Out1) -> To Workspace111/1
  [in1] -> M113/1(DW1)
  [in2] -> M113/2(DW2)
  [in3] -> M113/3(DW3)
  [in5] -> M113/4(P1W2)
  [in6] -> M113/5(P2W3)
  [in10] -> M113/6(O1)
  [in11] -> M113/7(O2)
  [in12] -> M113/8(O3)
  [in17] -> M113/9(CW3C)
  M113/1(W1Pos) -> Eval112/1(In1)
  M113/2(W2Pos) -> Eval112/2(In2)
  M113/3(W3Pos) -> Eval112/3(In3)
  Eval112/1(Out1) -> To Workspace112/1
  [in1] -> M115/1(DW1)
  [in2] -> M115/2(DW2)
  [in3] -> M115/3(DW3)
  [in5] -> M115/4(P1W2)
  [in6] -> M115/5(P2W3)
  [in10] -> M115/6(O1)
  [in11] -> M115/7(O2)
  [in12] -> M115/8(O3)
  [in17] -> M115/9(CW3C)
  M115/1(W1Pos) -> Eval114/1(In1)
  M115/2(W2Pos) -> Eval114/2(In2)
  M115/3(W3Pos) -> Eval114/3(In3)
  Eval114/1(Out1) -> To Workspace114/1
  [in1] -> M116/1(DW1)
  [in2] -> M116/2(DW2)
  [in3] -> M116/3(DW3)
  [in5] -> M116/4(P1W2)
  [in6] -> M116/5(P2W3)
  [in10] -> M116/6(O1)
  [in11] -> M116/7(O2)
  [in12] -> M116/8(O3)
  [in17] -> M116/9(CW3C)
  M116/1(W1Pos) -> Eval115/1(In1)
  M116/2(W2Pos) -> Eval115/2(In2)
  M116/3(W3Pos) -> Eval115/3(In3)
  Eval115/1(Out1) -> To Workspace115/1
  [in1] -> M117/1(DW1)
  [in2] -> M117/2(DW2)
  [in3] -> M117/3(DW3)
  [in5] -> M117/4(P1W2)
  [in6] -> M117/5(P2W3)
  [in10] -> M117/6(O1)
  [in11] -> M117/7(O2)
  [in12] -> M117/8(O3)
  [in17] -> M117/9(CW3C)
  M117/1(W1Pos) -> Eval116/1(In1)
  M117/2(W2Pos) -> Eval116/2(In2)
  M117/3(W3Pos) -> Eval116/3(In3)
  Eval116/1(Out1) -> To Workspace116/1
  [in1] -> M119/1(DW1)
  [in2] -> M119/2(DW2)
  [in3] -> M119/3(DW3)
  [in5] -> M119/4(P1W2)
  [in6] -> M119/5(P2W3)
  [in10] -> M119/6(O1)
  [in11] -> M119/7(O2)
  [in12] -> M119/8(O3)
  [in17] -> M119/9(CW3C)
  M119/1(W1Pos) -> Eval118/1(In1)
  M119/2(W2Pos) -> Eval118/2(In2)
  M119/3(W3Pos) -> Eval118/3(In3)
  Eval118/1(Out1) -> To Workspace118/1
  [in1] -> M120/1(DW1)
  [in2] -> M120/2(DW2)
  [in3] -> M120/3(DW3)
  [in5] -> M120/4(P1W2)
  [in6] -> M120/5(P2W3)
  [in10] -> M120/6(O1)
  [in11] -> M120/7(O2)
  [in12] -> M120/8(O3)
  [in17] -> M120/9(CW3C)
  M120/1(W1Pos) -> Eval119/1(In1)
  M120/2(W2Pos) -> Eval119/2(In2)
  M120/3(W3Pos) -> Eval119/3(In3)
  Eval119/1(Out1) -> To Workspace119/1
  [in1] -> M121/1(DW1)
  [in2] -> M121/2(DW2)
  [in3] -> M121/3(DW3)
  [in5] -> M121/4(P1W2)
  [in6] -> M121/5(P2W3)
  [in10] -> M121/6(O1)
  [in11] -> M121/7(O2)
  [in12] -> M121/8(O3)
  [in17] -> M121/9(CW3C)
  M121/1(W1Pos) -> Eval120/1(In1)
  M121/2(W2Pos) -> Eval120/2(In2)
  M121/3(W3Pos) -> Eval120/3(In3)
  Eval120/1(Out1) -> To Workspace120/1
  [in1] -> M123/1(DW1)
  [in2] -> M123/2(DW2)
  [in3] -> M123/3(DW3)
  [in5] -> M123/4(P1W2)
  [in6] -> M123/5(P2W3)
  [in10] -> M123/6(O1)
  [in11] -> M123/7(O2)
  [in12] -> M123/8(O3)
  [in17] -> M123/9(CW3C)
  M123/1(W1Pos) -> Eval122/1(In1)
  M123/2(W2Pos) -> Eval122/2(In2)
  M123/3(W3Pos) -> Eval122/3(In3)
  Eval122/1(Out1) -> To Workspace122/1
  [in1] -> M124/1(DW1)
  [in2] -> M124/2(DW2)
  [in3] -> M124/3(DW3)
  [in5] -> M124/4(P1W2)
  [in6] -> M124/5(P2W3)
  [in10] -> M124/6(O1)
  [in11] -> M124/7(O2)
  [in12] -> M124/8(O3)
  [in17] -> M124/9(CW3C)
  M124/1(W1Pos) -> Eval123/1(In1)
  M124/2(W2Pos) -> Eval123/2(In2)
  M124/3(W3Pos) -> Eval123/3(In3)
  Eval123/1(Out1) -> To Workspace123/1
  [in1] -> M125/1(DW1)
  [in2] -> M125/2(DW2)
  [in3] -> M125/3(DW3)
  [in5] -> M125/4(P1W2)
  [in6] -> M125/5(P2W3)
  [in10] -> M125/6(O1)
  [in11] -> M125/7(O2)
  [in12] -> M125/8(O3)
  [in17] -> M125/9(CW3C)
  M125/1(W1Pos) -> Eval124/1(In1)
  M125/2(W2Pos) -> Eval124/2(In2)
  M125/3(W3Pos) -> Eval124/3(In3)
  Eval124/1(Out1) -> To Workspace124/1
  [in1] -> M127/1(DW1)
  [in2] -> M127/2(DW2)
  [in3] -> M127/3(DW3)
  [in5] -> M127/4(P1W2)
  [in6] -> M127/5(P2W3)
  [in10] -> M127/6(O1)
  [in11] -> M127/7(O2)
  [in12] -> M127/8(O3)
  [in17] -> M127/9(CW3C)
  M127/1(W1Pos) -> Eval126/1(In1)
  M127/2(W2Pos) -> Eval126/2(In2)
  M127/3(W3Pos) -> Eval126/3(In3)
  Eval126/1(Out1) -> To Workspace126/1
  [in1] -> M128/1(DW1)
  [in2] -> M128/2(DW2)
  [in3] -> M128/3(DW3)
  [in5] -> M128/4(P1W2)
  [in6] -> M128/5(P2W3)
  [in10] -> M128/6(O1)
  [in11] -> M128/7(O2)
  [in12] -> M128/8(O3)
  [in17] -> M128/9(CW3C)
  M128/1(W1Pos) -> Eval127/1(In1)
  M128/2(W2Pos) -> Eval127/2(In2)
  M128/3(W3Pos) -> Eval127/3(In3)
  Eval127/1(Out1) -> To Workspace127/1
  [in1] -> M129/1(DW1)
  [in2] -> M129/2(DW2)
  [in3] -> M129/3(DW3)
  [in5] -> M129/4(P1W2)
  [in6] -> M129/5(P2W3)
  [in10] -> M129/6(O1)
  [in11] -> M129/7(O2)
  [in12] -> M129/8(O3)
  [in17] -> M129/9(CW3C)
  M129/1(W1Pos) -> Eval128/1(In1)
  M129/2(W2Pos) -> Eval128/2(In2)
  M129/3(W3Pos) -> Eval128/3(In3)
  Eval128/1(Out1) -> To Workspace128/1
  [in1] -> M131/1(DW1)
  [in2] -> M131/2(DW2)
  [in3] -> M131/3(DW3)
  [in5] -> M131/4(P1W2)
  [in6] -> M131/5(P2W3)
  [in10] -> M131/6(O1)
  [in11] -> M131/7(O2)
  [in12] -> M131/8(O3)
  [in17] -> M131/9(CW3C)
  M131/1(W1Pos) -> Eval130/1(In1)
  M131/2(W2Pos) -> Eval130/2(In2)
  M131/3(W3Pos) -> Eval130/3(In3)
  Eval130/1(Out1) -> To Workspace130/1
  [in1] -> M132/1(DW1)
  [in2] -> M132/2(DW2)
  [in3] -> M132/3(DW3)
  [in5] -> M132/4(P1W2)
  [in6] -> M132/5(P2W3)
  [in10] -> M132/6(O1)
  [in11] -> M132/7(O2)
  [in12] -> M132/8(O3)
  [in17] -> M132/9(CW3C)
  M132/1(W1Pos) -> Eval131/1(In1)
  M132/2(W2Pos) -> Eval131/2(In2)
  M132/3(W3Pos) -> Eval131/3(In3)
  Eval131/1(Out1) -> To Workspace131/1
  [in1] -> M133/1(DW1)
  [in2] -> M133/2(DW2)
  [in3] -> M133/3(DW3)
  [in5] -> M133/4(P1W2)
  [in6] -> M133/5(P2W3)
  [in10] -> M133/6(O1)
  [in11] -> M133/7(O2)
  [in12] -> M133/8(O3)
  [in17] -> M133/9(CW3C)
  M133/1(W1Pos) -> Eval132/1(In1)
  M133/2(W2Pos) -> Eval132/2(In2)
  M133/3(W3Pos) -> Eval132/3(In3)
  Eval132/1(Out1) -> To Workspace132/1
  [in1] -> M135/1(DW1)
  [in2] -> M135/2(DW2)
  [in3] -> M135/3(DW3)
  [in5] -> M135/4(P1W2)
  [in6] -> M135/5(P2W3)
  [in10] -> M135/6(O1)
  [in11] -> M135/7(O2)
  [in12] -> M135/8(O3)
  [in17] -> M135/9(CW3C)
  M135/1(W1Pos) -> Eval134/1(In1)
  M135/2(W2Pos) -> Eval134/2(In2)
  M135/3(W3Pos) -> Eval134/3(In3)
  Eval134/1(Out1) -> To Workspace134/1
  [in1] -> M136/1(DW1)
  [in2] -> M136/2(DW2)
  [in3] -> M136/3(DW3)
  [in5] -> M136/4(P1W2)
  [in6] -> M136/5(P2W3)
  [in10] -> M136/6(O1)
  [in11] -> M136/7(O2)
  [in12] -> M136/8(O3)
  [in17] -> M136/9(CW3C)
  M136/1(W1Pos) -> Eval135/1(In1)
  M136/2(W2Pos) -> Eval135/2(In2)
  M136/3(W3Pos) -> Eval135/3(In3)
  Eval135/1(Out1) -> To Workspace135/1
  [in1] -> M137/1(DW1)
  [in2] -> M137/2(DW2)
  [in3] -> M137/3(DW3)
  [in5] -> M137/4(P1W2)
  [in6] -> M137/5(P2W3)
  [in10] -> M137/6(O1)
  [in11] -> M137/7(O2)
  [in12] -> M137/8(O3)
  [in17] -> M137/9(CW3C)
  M137/1(W1Pos) -> Eval136/1(In1)
  M137/2(W2Pos) -> Eval136/2(In2)
  M137/3(W3Pos) -> Eval136/3(In3)
  Eval136/1(Out1) -> To Workspace136/1
  [in1] -> M139/1(DW1)
  [in2] -> M139/2(DW2)
  [in3] -> M139/3(DW3)
  [in5] -> M139/4(P1W2)
  [in6] -> M139/5(P2W3)
  [in10] -> M139/6(O1)
  [in11] -> M139/7(O2)
  [in12] -> M139/8(O3)
  [in17] -> M139/9(CW3C)
  M139/1(W1Pos) -> Eval138/1(In1)
  M139/2(W2Pos) -> Eval138/2(In2)
  M139/3(W3Pos) -> Eval138/3(In3)
  Eval138/1(Out1) -> To Workspace138/1
  [in1] -> M140/1(DW1)
  [in2] -> M140/2(DW2)
  [in3] -> M140/3(DW3)
  [in5] -> M140/4(P1W2)
  [in6] -> M140/5(P2W3)
  [in10] -> M140/6(O1)
  [in11] -> M140/7(O2)
  [in12] -> M140/8(O3)
  [in17] -> M140/9(CW3C)
  M140/1(W1Pos) -> Eval139/1(In1)
  M140/2(W2Pos) -> Eval139/2(In2)
  M140/3(W3Pos) -> Eval139/3(In3)
  Eval139/1(Out1) -> To Workspace139/1
  [in1] -> M141/1(DW1)
  [in2] -> M141/2(DW2)
  [in3] -> M141/3(DW3)
  [in5] -> M141/4(P1W2)
  [in6] -> M141/5(P2W3)
  [in10] -> M141/6(O1)
  [in11] -> M141/7(O2)
  [in12] -> M141/8(O3)
  [in17] -> M141/9(CW3C)
  M141/1(W1Pos) -> Eval140/1(In1)
  M141/2(W2Pos) -> Eval140/2(In2)
  M141/3(W3Pos) -> Eval140/3(In3)
  Eval140/1(Out1) -> To Workspace140/1
  [in1] -> M143/1(DW1)
  [in2] -> M143/2(DW2)
  [in3] -> M143/3(DW3)
  [in5] -> M143/4(P1W2)
  [in6] -> M143/5(P2W3)
  [in10] -> M143/6(O1)
  [in11] -> M143/7(O2)
  [in12] -> M143/8(O3)
  [in17] -> M143/9(CW3C)
  M143/1(W1Pos) -> Eval142/1(In1)
  M143/2(W2Pos) -> Eval142/2(In2)
  M143/3(W3Pos) -> Eval142/3(In3)
  Eval142/1(Out1) -> To Workspace142/1
  [in1] -> M144/1(DW1)
  [in2] -> M144/2(DW2)
  [in3] -> M144/3(DW3)
  [in5] -> M144/4(P1W2)
  [in6] -> M144/5(P2W3)
  [in10] -> M144/6(O1)
  [in11] -> M144/7(O2)
  [in12] -> M144/8(O3)
  [in17] -> M144/9(CW3C)
  M144/1(W1Pos) -> Eval143/1(In1)
  M144/2(W2Pos) -> Eval143/2(In2)
  M144/3(W3Pos) -> Eval143/3(In3)
  Eval143/1(Out1) -> To Workspace143/1
  [in1] -> M145/1(DW1)
  [in2] -> M145/2(DW2)
  [in3] -> M145/3(DW3)
  [in5] -> M145/4(P1W2)
  [in6] -> M145/5(P2W3)
  [in10] -> M145/6(O1)
  [in11] -> M145/7(O2)
  [in12] -> M145/8(O3)
  [in17] -> M145/9(CW3C)
  M145/1(W1Pos) -> Eval144/1(In1)
  M145/2(W2Pos) -> Eval144/2(In2)
  M145/3(W3Pos) -> Eval144/3(In3)
  Eval144/1(Out1) -> To Workspace144/1
  [in1] -> M147/1(DW1)
  [in2] -> M147/2(DW2)
  [in3] -> M147/3(DW3)
  [in5] -> M147/4(P1W2)
  [in6] -> M147/5(P2W3)
  [in10] -> M147/6(O1)
  [in11] -> M147/7(O2)
  [in12] -> M147/8(O3)
  [in17] -> M147/9(CW3C)
  M147/1(W1Pos) -> Eval146/1(In1)
  M147/2(W2Pos) -> Eval146/2(In2)
  M147/3(W3Pos) -> Eval146/3(In3)
  Eval146/1(Out1) -> To Workspace146/1
  [in1] -> M148/1(DW1)
  [in2] -> M148/2(DW2)
  [in3] -> M148/3(DW3)
  [in5] -> M148/4(P1W2)
  [in6] -> M148/5(P2W3)
  [in10] -> M148/6(O1)
  [in11] -> M148/7(O2)
  [in12] -> M148/8(O3)
  [in17] -> M148/9(CW3C)
  M148/1(W1Pos) -> Eval147/1(In1)
  M148/2(W2Pos) -> Eval147/2(In2)
  M148/3(W3Pos) -> Eval147/3(In3)
  Eval147/1(Out1) -> To Workspace147/1
  [in1] -> M149/1(DW1)
  [in2] -> M149/2(DW2)
  [in3] -> M149/3(DW3)
  [in5] -> M149/4(P1W2)
  [in6] -> M149/5(P2W3)
  [in10] -> M149/6(O1)
  [in11] -> M149/7(O2)
  [in12] -> M149/8(O3)
  [in17] -> M149/9(CW3C)
  M149/1(W1Pos) -> Eval148/1(In1)
  M149/2(W2Pos) -> Eval148/2(In2)
  M149/3(W3Pos) -> Eval148/3(In3)
  Eval148/1(Out1) -> To Workspace148/1
  [in1] -> M151/1(DW1)
  [in2] -> M151/2(DW2)
  [in3] -> M151/3(DW3)
  [in5] -> M151/4(P1W2)
  [in6] -> M151/5(P2W3)
  [in10] -> M151/6(O1)
  [in11] -> M151/7(O2)
  [in12] -> M151/8(O3)
  [in17] -> M151/9(CW3C)
  M151/1(W1Pos) -> Eval150/1(In1)
  M151/2(W2Pos) -> Eval150/2(In2)
  M151/3(W3Pos) -> Eval150/3(In3)
  Eval150/1(Out1) -> To Workspace150/1
  [in1] -> M152/1(DW1)
  [in2] -> M152/2(DW2)
  [in3] -> M152/3(DW3)
  [in5] -> M152/4(P1W2)
  [in6] -> M152/5(P2W3)
  [in10] -> M152/6(O1)
  [in11] -> M152/7(O2)
  [in12] -> M152/8(O3)
  [in17] -> M152/9(CW3C)
  M152/1(W1Pos) -> Eval151/1(In1)
  M152/2(W2Pos) -> Eval151/2(In2)
  M152/3(W3Pos) -> Eval151/3(In3)
  Eval151/1(Out1) -> To Workspace151/1
  [in1] -> M153/1(DW1)
  [in2] -> M153/2(DW2)
  [in3] -> M153/3(DW3)
  [in5] -> M153/4(P1W2)
  [in6] -> M153/5(P2W3)
  [in10] -> M153/6(O1)
  [in11] -> M153/7(O2)
  [in12] -> M153/8(O3)
  [in17] -> M153/9(CW3C)
  M153/1(W1Pos) -> Eval152/1(In1)
  M153/2(W2Pos) -> Eval152/2(In2)
  M153/3(W3Pos) -> Eval152/3(In3)
  Eval152/1(Out1) -> To Workspace152/1
  [in1] -> M155/1(DW1)
  [in2] -> M155/2(DW2)
  [in3] -> M155/3(DW3)
  [in5] -> M155/4(P1W2)
  [in6] -> M155/5(P2W3)
  [in10] -> M155/6(O1)
  [in11] -> M155/7(O2)
  [in12] -> M155/8(O3)
  [in17] -> M155/9(CW3C)
  M155/1(W1Pos) -> Eval154/1(In1)
  M155/2(W2Pos) -> Eval154/2(In2)
  M155/3(W3Pos) -> Eval154/3(In3)
  Eval154/1(Out1) -> To Workspace154/1
  [in1] -> M156/1(DW1)
  [in2] -> M156/2(DW2)
  [in3] -> M156/3(DW3)
  [in5] -> M156/4(P1W2)
  [in6] -> M156/5(P2W3)
  [in10] -> M156/6(O1)
  [in11] -> M156/7(O2)
  [in12] -> M156/8(O3)
  [in17] -> M156/9(CW3C)
  M156/1(W1Pos) -> Eval155/1(In1)
  M156/2(W2Pos) -> Eval155/2(In2)
  M156/3(W3Pos) -> Eval155/3(In3)
  Eval155/1(Out1) -> To Workspace155/1
  [in1] -> M157/1(DW1)
  [in2] -> M157/2(DW2)
  [in3] -> M157/3(DW3)
  [in5] -> M157/4(P1W2)
  [in6] -> M157/5(P2W3)
  [in10] -> M157/6(O1)
  [in11] -> M157/7(O2)
  [in12] -> M157/8(O3)
  [in17] -> M157/9(CW3C)
  M157/1(W1Pos) -> Eval156/1(In1)
  M157/2(W2Pos) -> Eval156/2(In2)
  M157/3(W3Pos) -> Eval156/3(In3)
  Eval156/1(Out1) -> To Workspace156/1
  [in1] -> M159/1(DW1)
  [in2] -> M159/2(DW2)
  [in3] -> M159/3(DW3)
  [in5] -> M159/4(P1W2)
  [in6] -> M159/5(P2W3)
  [in10] -> M159/6(O1)
  [in11] -> M159/7(O2)
  [in12] -> M159/8(O3)
  [in17] -> M159/9(CW3C)
  M159/1(W1Pos) -> Eval158/1(In1)
  M159/2(W2Pos) -> Eval158/2(In2)
  M159/3(W3Pos) -> Eval158/3(In3)
  Eval158/1(Out1) -> To Workspace158/1
  [in1] -> M160/1(DW1)
  [in2] -> M160/2(DW2)
  [in3] -> M160/3(DW3)
  [in5] -> M160/4(P1W2)
  [in6] -> M160/5(P2W3)
  [in10] -> M160/6(O1)
  [in11] -> M160/7(O2)
  [in12] -> M160/8(O3)
  [in17] -> M160/9(CW3C)
  M160/1(W1Pos) -> Eval159/1(In1)
  M160/2(W2Pos) -> Eval159/2(In2)
  M160/3(W3Pos) -> Eval159/3(In3)
  Eval159/1(Out1) -> To Workspace159/1
  [in1] -> M161/1(DW1)
  [in2] -> M161/2(DW2)
  [in3] -> M161/3(DW3)
  [in5] -> M161/4(P1W2)
  [in6] -> M161/5(P2W3)
  [in10] -> M161/6(O1)
  [in11] -> M161/7(O2)
  [in12] -> M161/8(O3)
  [in17] -> M161/9(CW3C)
  M161/1(W1Pos) -> Eval160/1(In1)
  M161/2(W2Pos) -> Eval160/2(In2)
  M161/3(W3Pos) -> Eval160/3(In3)
  Eval160/1(Out1) -> To Workspace160/1
  [in1] -> M163/1(DW1)
  [in2] -> M163/2(DW2)
  [in3] -> M163/3(DW3)
  [in5] -> M163/4(P1W2)
  [in6] -> M163/5(P2W3)
  [in10] -> M163/6(O1)
  [in11] -> M163/7(O2)
  [in12] -> M163/8(O3)
  [in17] -> M163/9(CW3C)
  M163/1(W1Pos) -> Eval162/1(In1)
  M163/2(W2Pos) -> Eval162/2(In2)
  M163/3(W3Pos) -> Eval162/3(In3)
  Eval162/1(Out1) -> To Workspace162/1
  [in1] -> M164/1(DW1)
  [in2] -> M164/2(DW2)
  [in3] -> M164/3(DW3)
  [in5] -> M164/4(P1W2)
  [in6] -> M164/5(P2W3)
  [in10] -> M164/6(O1)
  [in11] -> M164/7(O2)
  [in12] -> M164/8(O3)
  [in17] -> M164/9(CW3C)
  M164/1(W1Pos) -> Eval163/1(In1)
  M164/2(W2Pos) -> Eval163/2(In2)
  M164/3(W3Pos) -> Eval163/3(In3)
  Eval163/1(Out1) -> To Workspace163/1
  [in1] -> M165/1(DW1)
  [in2] -> M165/2(DW2)
  [in3] -> M165/3(DW3)
  [in5] -> M165/4(P1W2)
  [in6] -> M165/5(P2W3)
  [in10] -> M165/6(O1)
  [in11] -> M165/7(O2)
  [in12] -> M165/8(O3)
  [in17] -> M165/9(CW3C)
  M165/1(W1Pos) -> Eval164/1(In1)
  M165/2(W2Pos) -> Eval164/2(In2)
  M165/3(W3Pos) -> Eval164/3(In3)
  Eval164/1(Out1) -> To Workspace164/1
  [in1] -> M167/1(DW1)
  [in2] -> M167/2(DW2)
  [in3] -> M167/3(DW3)
  [in5] -> M167/4(P1W2)
  [in6] -> M167/5(P2W3)
  [in10] -> M167/6(O1)
  [in11] -> M167/7(O2)
  [in12] -> M167/8(O3)
  [in17] -> M167/9(CW3C)
  M167/1(W1Pos) -> Eval166/1(In1)
  M167/2(W2Pos) -> Eval166/2(In2)
  M167/3(W3Pos) -> Eval166/3(In3)
  Eval166/1(Out1) -> To Workspace166/1
  [in1] -> M168/1(DW1)
  [in2] -> M168/2(DW2)
  [in3] -> M168/3(DW3)
  [in5] -> M168/4(P1W2)
  [in6] -> M168/5(P2W3)
  [in10] -> M168/6(O1)
  [in11] -> M168/7(O2)
  [in12] -> M168/8(O3)
  [in17] -> M168/9(CW3C)
  M168/1(W1Pos) -> Eval167/1(In1)
  M168/2(W2Pos) -> Eval167/2(In2)
  M168/3(W3Pos) -> Eval167/3(In3)
  Eval167/1(Out1) -> To Workspace167/1
  [in1] -> M169/1(DW1)
  [in2] -> M169/2(DW2)
  [in3] -> M169/3(DW3)
  [in5] -> M169/4(P1W2)
  [in6] -> M169/5(P2W3)
  [in10] -> M169/6(O1)
  [in11] -> M169/7(O2)
  [in12] -> M169/8(O3)
  [in17] -> M169/9(CW3C)
  M169/1(W1Pos) -> Eval168/1(In1)
  M169/2(W2Pos) -> Eval168/2(In2)
  M169/3(W3Pos) -> Eval168/3(In3)
  Eval168/1(Out1) -> To Workspace168/1
  [in1] -> M171/1(DW1)
  [in2] -> M171/2(DW2)
  [in3] -> M171/3(DW3)
  [in5] -> M171/4(P1W2)
  [in6] -> M171/5(P2W3)
  [in10] -> M171/6(O1)
  [in11] -> M171/7(O2)
  [in12] -> M171/8(O3)
  [in17] -> M171/9(CW3C)
  M171/1(W1Pos) -> Eval170/1(In1)
  M171/2(W2Pos) -> Eval170/2(In2)
  M171/3(W3Pos) -> Eval170/3(In3)
  Eval170/1(Out1) -> To Workspace170/1
  [in1] -> M172/1(DW1)
  [in2] -> M172/2(DW2)
  [in3] -> M172/3(DW3)
  [in5] -> M172/4(P1W2)
  [in6] -> M172/5(P2W3)
  [in10] -> M172/6(O1)
  [in11] -> M172/7(O2)
  [in12] -> M172/8(O3)
  [in17] -> M172/9(CW3C)
  M172/1(W1Pos) -> Eval171/1(In1)
  M172/2(W2Pos) -> Eval171/2(In2)
  M172/3(W3Pos) -> Eval171/3(In3)
  Eval171/1(Out1) -> To Workspace171/1
  [in1] -> M173/1(DW1)
  [in2] -> M173/2(DW2)
  [in3] -> M173/3(DW3)
  [in5] -> M173/4(P1W2)
  [in6] -> M173/5(P2W3)
  [in10] -> M173/6(O1)
  [in11] -> M173/7(O2)
  [in12] -> M173/8(O3)
  [in17] -> M173/9(CW3C)
  M173/1(W1Pos) -> Eval172/1(In1)
  M173/2(W2Pos) -> Eval172/2(In2)
  M173/3(W3Pos) -> Eval172/3(In3)
  Eval172/1(Out1) -> To Workspace172/1
  Inputs/1(DW1) -> dtc_DW1/1
  dtc_DW1/1 -> CPSUT/1(DW1), [in1]
  Inputs/2(DW2) -> dtc_DW2/1
  dtc_DW2/1 -> CPSUT/2(DW2), [in2]
  Inputs/3(DW3) -> dtc_DW3/1
  dtc_DW3/1 -> CPSUT/3(DW3), [in3]
  Inputs/4(P1W2) -> dtc_P1W2/1
  dtc_P1W2/1 -> CPSUT/4(P1W2), [in5]
  Inputs/5(P2W3) -> dtc_P2W3/1
  dtc_P2W3/1 -> CPSUT/5(P2W3), [in6]
  Inputs/6(O1) -> dtc_O1/1
  dtc_O1/1 -> CPSUT/6(O1), [in10]
  Inputs/7(O2) -> dtc_O2/1
  dtc_O2/1 -> CPSUT/7(O2), [in11]
  Inputs/8(O3) -> dtc_O3/1
  dtc_O3/1 -> CPSUT/8(O3), [in12]
  Inputs/9(CW3C) -> dtc_CW3C/1
  dtc_CW3C/1 -> CPSUT/9(CW3C), [in17]
